simulink model "gm_Copy_of_uz_pmsm_model_9ph_21b_all_double"  (R2022a)
settings: Solver=FixedStepAuto  StartTime=0.0  StopTime=0.8  RelTol=1e-3
PreLoadFcn:
  | uz_pmsm_model_9ph_init_parameter
undefined symbols (not defined in the file or in its folder): a, b, c, friction_coefficient, inertia, k_i_d, k_i_q, k_p_d, k_p_q, Kpd, L_d, L_o1, L_o2, L_q, L_x1, L_x2, L_y1, L_y2, L_zero, polepair, psi_pm, R_1, static_friction_torque, Tnd, ts
libraries: hdlsllib x90, hdlmdlgenlib x21, slpidlib x2, simulink x2, spsAlphaBetaZerotodq0Lib x1, pid_lib x1, spsdq0toAlphaBetaZeroLib x1
(part 2 of 3)

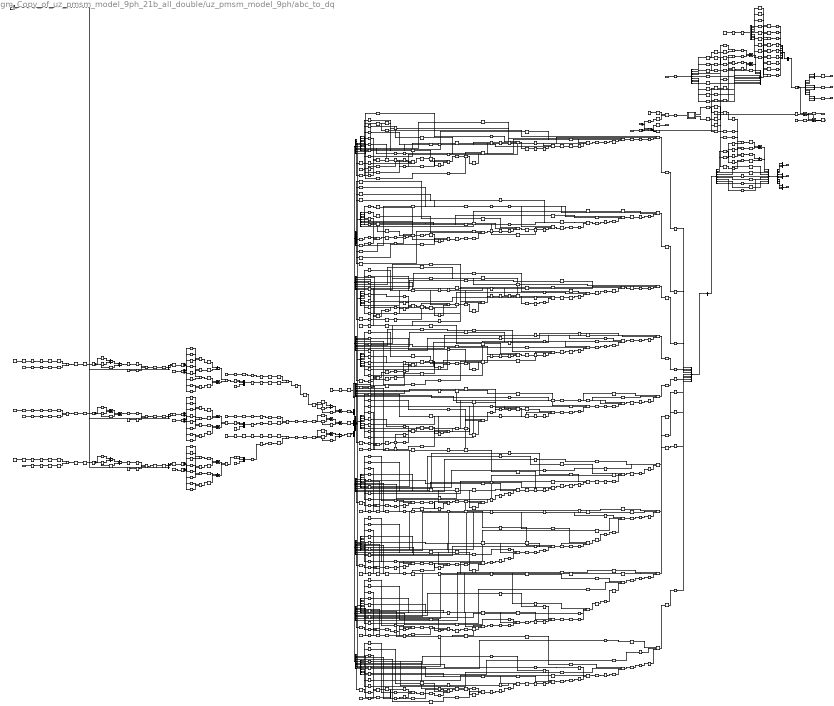
== system gm_Copy_of_uz_pmsm_model_9ph_21b_all_double/uz_pmsm_model_9ph/abc_to_dq ==
  current_in_dq : Inport  OutDataTypeStr=fixdt(1, 25, 12)  PortDimensions=[9]  SampleTime=1e-08
  theta_el1 : Inport  Port=2  OutDataTypeStr=fixdt(1, 18, 14)  PortDimensions=1  SampleTime=1e-08
  trigger_new_values : Inport  Port=3  OutDataTypeStr=boolean  PortDimensions=1  SampleTime=1e-08
  u_abc1_pl : Inport  Port=4  OutDataTypeStr=fixdt(1, 25, 12)  PortDimensions=[3]  SampleTime=1e-08
  u_abc2_pl : Inport  Port=5  OutDataTypeStr=fixdt(1, 25, 12)  PortDimensions=[3]  SampleTime=1e-08
  u_abc3_pl : Inport  Port=6  OutDataTypeStr=fixdt(1, 25, 12)  PortDimensions=[3]  SampleTime=1e-08
  Add : Sum  AccumDataTypeStr=fixdt(1, 26, 12)  OutDataTypeStr=fixdt(1, 25, 12)  SampleTime=1e-08
  Add1 : Sum  Inputs=+-  AccumDataTypeStr=fixdt(1, 26, 12)  OutDataTypeStr=fixdt(1, 25, 12)  SampleTime=1e-08
  Add11 : Sum  AccumDataTypeStr=fixdt(1, 26, 12)  OutDataTypeStr=fixdt(1, 25, 12)  SampleTime=1e-08
  Add2 : Sum  Inputs=+-  AccumDataTypeStr=fixdt(1, 26, 12)  OutDataTypeStr=fixdt(1, 25, 12)  SampleTime=1e-08
  Complex to Real-Imag : ComplexToRealImag  SampleTime=1e-08
  Complex to Real-Imag1 : ComplexToRealImag  SampleTime=1e-08
  Complex to Real-Imag2 : ComplexToRealImag  SampleTime=1e-08
  Constant : Constant  Value=0  OutDataTypeStr=fixdt(1, 25, 12)  SampleTime=1e-08
  Constant1 : Constant  Value="fi(0,1,18,16,\"hex\",\"08000 + 3b619 i\")"  OutDataTypeStr=fixdt(1, 18, 16)  SampleTime=1e-08
  Constant11 : Constant  Value="fi(0,1,18,16,\"hex\",\"08000 + 3b619 i\")"  OutDataTypeStr=fixdt(1, 18, 16)  SampleTime=1e-08
  Constant12 : Constant  Value="fi(0,1,18,16,\"hex\",\"08000 + 3b619 i\")"  OutDataTypeStr=fixdt(1, 18, 16)  SampleTime=1e-08
  Constant13 : Constant  Value=[0.22222137451171875;0;0.22222137451171875;0;0.22222137451171875;0;0.22222137451171875;0;0.111114501953125;-0.111114501953125;0.19245147705078125;0.22222137451171875;0;-0.111114501953125;-0.19245147705078125;-0.111114501953125;0.19245147705078125;0.111114501953125;-0.111114501953125;-0.19245147705078125;0.22222137451171875;0;-0.111114501953125;0.19245147705078125;-0.111114501953125;-0.19245147705078125;0.111114501953125;0.20882415771484375;0.0760040283203125;0.111114501953125;0.19245147705078125;-0.0385894775390625;0.21884918212890625;-0.17023468017578125;0.14284515380859375;-0.111114501953125;-0.17023468017578125;0.14284515380859375;0.111114501953125;0.19245147705078125;0.20882415771484375;-0.0760040283203125;-0.0385894775390625;-0.21884918212890625;-0.111114501953125;-0.0385894775390625;-0.21884918212890625;0.111114501953125;0.19245147705078125;-0.17023468017578125;-0.14284515380859375;0.20882415771484375;0.0760040283203125;-0.111114501953125;0.17023468017578125;0.14284515380859375;-0.111114501953125;0.19245147705078125;-0.20882415771484375;-0.0760040283203125;0.0385894775390625;-0.21884918212890625;0.111114501953125;-0.20882415771484375;0.0760040283203125;-0.111114501953125;0.19245147705078125;0.0385894775390625;0.21884918212890625;0.17023468017578125;0.14284515380859375;0.111114501953125;0.0385894775390625;-0.21884918212890625;-0.111114501953125;0.19245147705078125;0.17023468017578125;-0.14284515380859375;-0.20882415771484375;0.0760040283203125;0.111114501953125]  OutDataTypeStr=fixdt(1, 18, 17)  SampleTime=1e-08
  Constant14 : Constant  Value=[1;-0.5;-0.5;0.939697265625;-0.7660369873046875;-0.17364501953125;0.7660369873046875;-0.939697265625;0.17364501953125;0;0.86602783203125;-0.86602783203125;0.3420257568359375;0.642791748046875;-0.98480224609375;0.642791748046875;0.3420257568359375;-0.98480224609375;1;1;1;0.5;0.5;0.5;-0.5;-0.5;-0.5;0;0;0;0.86602783203125;0.86602783203125;0.86602783203125;0.86602783203125;0.86602783203125;0.86602783203125;1;-0.5;-0.5;-0.17364501953125;0.939697265625;-0.7660369873046875;-0.939697265625;0.17364501953125;0.7660369873046875;0;-0.86602783203125;0.86602783203125;0.98480224609375;-0.3420257568359375;-0.642791748046875;-0.3420257568359375;0.98480224609375;-0.642791748046875;1;-0.5;-0.5;-0.7660369873046875;-0.17364501953125;0.939697265625;0.17364501953125;0.7660369873046875;-0.939697265625;0;0.86602783203125;-0.86602783203125;0.642791748046875;-0.98480224609375;0.3420257568359375;-0.98480224609375;0.642791748046875;0.3420257568359375;1;1;1;-1;-1;-1;1;1;1]  OutDataTypeStr=fixdt(1, 18, 16)  SampleTime=1e-08
  Constant2 : Constant  Value=0  OutDataTypeStr=fixdt(1, 25, 12)  SampleTime=1e-08
  Constant3 : Constant  Value=0  OutDataTypeStr=fixdt(1, 25, 12)  SampleTime=1e-08
  Data Type Conversion28 : DataTypeConversion  OutDataTypeStr=fixdt(1, 25, 12)  RndMeth=Nearest  SampleTime=1e-08  SaturateOnIntegerOverflow=off
  Data Type Conversion28_out1_0_wire : hdlmdlgenlib/Buffer
      settings: SourceProductBaseCode=SL
  Data Type Conversion28_out1_1_wire : hdlmdlgenlib/Buffer
      settings: SourceProductBaseCode=SL
  Delay1 : Delay  DelayLength=double(1)  InitialCondition=0  SampleTime=1e-08
  Delay2 : Delay  DelayLength=double(1)  InitialCondition=0  SampleTime=1e-08
  Delay9 : Delay  DelayLength=double(1)  InitialCondition=0  SampleTime=1e-08
  Delay9_enbsw : Switch  Criteria=u2 ~= 0  Threshold=double(0)  OutDataTypeStr=fixdt(1, 25, 12)  SampleTime=1e-08  SaturateOnIntegerOverflow=off  InputSameDT=off
  Demux1_mux_1 : Mux  Inputs=3
  Demux1_mux_2 : Mux  Inputs=3
  Demux1_mux_3 : Mux  Inputs=3
  Demux_mux_1 : Mux  Inputs=3
  Demux_mux_2 : Mux  Inputs=3
  Demux_mux_3 : Mux  Inputs=3
  Divide{,1..4,11,21,31} (8 alike) : Product  Inputs=**  OutDataTypeStr=fixdt(1, 25, 12)  SampleTime=1e-08
  From{1..2,11,17..18,21,171,181} (8 alike) : hdlmdlgenlib/Buffer
      settings: SourceProductBaseCode=SL
  Gain : Product  Inputs=**  OutDataTypeStr=fixdt(1, 18, 16)  SampleTime=1e-08
  Gain2 : Product  Inputs=**  OutDataTypeStr=fixdt(1, 43, 28)  SampleTime=1e-08
  Gain21 : Product  Inputs=**  OutDataTypeStr=fixdt(1, 43, 28)  SampleTime=1e-08
  Gain22 : Product  Inputs=**  OutDataTypeStr=fixdt(1, 43, 28)  SampleTime=1e-08
  Gain2_const : Constant  Value=0.6666717529296875  OutDataTypeStr=fixdt(1, 18, 16)  SampleTime=1e-08
  Gain2_const1 : Constant  Value=0.6666717529296875  OutDataTypeStr=fixdt(1, 18, 16)  SampleTime=1e-08
  Gain2_const2 : Constant  Value=0.6666717529296875  OutDataTypeStr=fixdt(1, 18, 16)  SampleTime=1e-08
  Gain2_out_dtc : DataTypeConversion  OutDataTypeStr=fixdt(1, 25, 12)  SampleTime=1e-08  RndMeth=Floor
  Gain2_out_dtc1 : DataTypeConversion  OutDataTypeStr=fixdt(1, 25, 12)  SampleTime=1e-08  RndMeth=Floor
  Gain2_out_dtc2 : DataTypeConversion  OutDataTypeStr=fixdt(1, 25, 12)  SampleTime=1e-08  RndMeth=Floor
  Gain4_const : Constant  Value=[1;0;0.5;-0.5;0.86602783203125;0.5;-0.5;-0.86602783203125;0.5]  OutDataTypeStr=fixdt(1, 18, 16)  SampleTime=1e-08
  Gain4_const1 : Constant  Value=[1;-0.5;-0.5;0;0.86602783203125;-0.86602783203125;1;1;1]  OutDataTypeStr=fixdt(1, 18, 16)  SampleTime=1e-08
  Gain4_const2 : Constant  Value=[1;0;0.5;-0.5;0.86602783203125;0.5;-0.5;-0.86602783203125;0.5]  OutDataTypeStr=fixdt(1, 18, 16)  SampleTime=1e-08
  Gain4_const3 : Constant  Value=[1;-0.5;-0.5;0;0.86602783203125;-0.86602783203125;1;1;1]  OutDataTypeStr=fixdt(1, 18, 16)  SampleTime=1e-08
  Gain4_const4 : Constant  Value=[1;0;0.5;-0.5;0.86602783203125;0.5;-0.5;-0.86602783203125;0.5]  OutDataTypeStr=fixdt(1, 18, 16)  SampleTime=1e-08
  Gain4_const5 : Constant  Value=[1;-0.5;-0.5;0;0.86602783203125;-0.86602783203125;1;1;1]  OutDataTypeStr=fixdt(1, 18, 16)  SampleTime=1e-08
  Gain_const : Constant  Value=0.1591548919677734375  OutDataTypeStr=fixdt(1, 18, 19)  SampleTime=1e-08
  Goto15 : hdlmdlgenlib/Buffer
      settings: SourceProductBaseCode=SL
  Goto16 : hdlmdlgenlib/Buffer
      settings: SourceProductBaseCode=SL
  HwModeRegister{,1..302} (303 alike) : Delay  DelayLength=double(1)  InitialCondition=0  SampleTime=1e-08
  MMul_add_01 : Sum  OutDataTypeStr=fixdt(1, 25, 12)  SaturateOnIntegerOverflow=on  SampleTime=1e-08
  MMul_add_011 : Sum  OutDataTypeStr=fixdt(1, 25, 12)  SaturateOnIntegerOverflow=on  SampleTime=1e-08
  MMul_add_012 : Sum  OutDataTypeStr=fixdt(1, 25, 12)  SaturateOnIntegerOverflow=on  SampleTime=1e-08
  MMul_add_013 : Sum  OutDataTypeStr=fixdt(1, 25, 12)  SaturateOnIntegerOverflow=on  SampleTime=1e-08
  MMul_add_014 : Sum  OutDataTypeStr=fixdt(1, 25, 12)  SaturateOnIntegerOverflow=on  SampleTime=1e-08
  MMul_add_015 : Sum  OutDataTypeStr=fixdt(1, 25, 12)  SaturateOnIntegerOverflow=on  SampleTime=1e-08
  MMul_add_{12,121..125} (6 alike) : Sum  OutDataTypeStr=fixdt(1, 25, 12)  SaturateOnIntegerOverflow=on  SampleTime=1e-08
  MMul_dot_product{,1..5} (6 alike) : Product  Inputs=**  OutDataTypeStr=fixdt(1, 43, 28)  SampleTime=1e-08
  MMul_dot_product_out_dtc{,1..5} (6 alike) : DataTypeConversion  OutDataTypeStr=fixdt(1, 25, 12)  SampleTime=1e-08  RndMeth=Floor
  MatrixMultiply_out1_0_wire : hdlmdlgenlib/Buffer
      settings: SourceProductBaseCode=SL
  MatrixMultiply_out1_1_wire : hdlmdlgenlib/Buffer
      settings: SourceProductBaseCode=SL
  PipelineRegister{,1..22,104..119} (39 alike) : Delay  DelayLength=double(1)  InitialCondition=0  SampleTime=1e-08
  PipelineRegister{23..103} (81 alike) : Delay  DelayLength=double(2)  InitialCondition=0  SampleTime=1e-08
  Product{,1..11} (12 alike) : Product  Inputs=**  OutDataTypeStr=fixdt(1, 25, 12)  SampleTime=1e-08
  Product_AC_minus_BD : Sum  Inputs=+-  OutDataTypeStr=fixdt(1, 25, 12)  SampleTime=1e-08
  Product_AC_minus_BD1 : Sum  Inputs=+-  OutDataTypeStr=fixdt(1, 25, 12)  SampleTime=1e-08
  Product_AC_minus_BD2 : Sum  Inputs=+-  OutDataTypeStr=fixdt(1, 25, 12)  SampleTime=1e-08
  Product_AD_plus_BC : Sum  OutDataTypeStr=fixdt(1, 25, 12)  SampleTime=1e-08
  Product_AD_plus_BC1 : Sum  OutDataTypeStr=fixdt(1, 25, 12)  SampleTime=1e-08
  Product_AD_plus_BC2 : Sum  OutDataTypeStr=fixdt(1, 25, 12)  SampleTime=1e-08
  Product_C2ReIm_{1..2,11..12,21..22} (6 alike) : ComplexToRealImag  SampleTime=1e-08
  Product_ReIm2Complex : RealImagToComplex  SampleTime=1e-08
  Product_ReIm2Complex1 : RealImagToComplex  SampleTime=1e-08
  Product_ReIm2Complex2 : RealImagToComplex  SampleTime=1e-08
  Real-Imag to Complex : RealImagToComplex  ConstantPart="fi(0,1,25,12,\"hex\",\"0000000\")"  SampleTime=1e-08
  Real-Imag to Complex1 : RealImagToComplex  ConstantPart="fi(0,1,25,12,\"hex\",\"0000000\")"  SampleTime=1e-08
  Real-Imag to Complex2 : RealImagToComplex  ConstantPart="fi(0,1,25,12,\"hex\",\"0000000\")"  SampleTime=1e-08
  Reshape{,1..5} (6 alike) : Reshape  OutputDimensionality=Column vector (2-D)
  Row2Col_in{0..1,11..15} (7 alike) : Reshape  OutputDimensionality=Column vector (2-D)
  Row2Col_in01 : Reshape  OutputDimensionality=Column vector (2-D)
  Row2Col_in02 : Reshape  OutputDimensionality=Column vector (2-D)
  Row2Col_in03 : Reshape  OutputDimensionality=Column vector (2-D)
  Row2Col_in04 : Reshape  OutputDimensionality=Column vector (2-D)
  Row2Col_in05 : Reshape  OutputDimensionality=Column vector (2-D)
  Sine HDL Optimized : Subsystem  mask(Sine and Cosine HDL optimized block){OutputFormula=sin(2*pi*u) and cos(2*pi*u), NumDataPoints=double(64), TableDataTypeStr=fixdt(0,16,15), SimulateLUTROMDelay=off}
      mask prompts: OutputFormula "Simulink:masks:OutputFormula_MP"; NumDataPoints "HDLShared:hdlshared:CosineHDL_Npts"; TableDataTypeStr "Simulink:blkprm_prompts:TABLE_UNIFIEDDATATYPE"; SimulateLUTROMDelay "HDLShared:hdlshared:CosineHDL_SimulateLUTDelay"
      mask help: Sine and Cosine HDL optimized block using quarter wave symmetry, and HDL friendly settings.
      mask Help: helpview([docroot '/hdlcoder/helptargets.map'],'SineAndCosineHDL_Optimized');
      mask TypeOptions OutputFormula: sin(2*pi*u) | cos(2*pi*u) | exp(j*2*pi*u) | sin(2*pi*u) and cos(2*pi*u)
      mask Display:
      | port_label('input',1,'u')
      | port_label('output',1,'sin(2*pi*u)')
      | port_label('output',2,'cos(2*pi*u)')
      | xpos = 0.35;
      | yoffset = 0.5;
      | if ( SimulateLUTROMDelay )
      |   text(xpos,yoffset,'HDL (Z^{-1})','texmode','on')
      | else
      |    text(xpos,yoffset,'HDL')
      | end
  Switch : Switch  Criteria=u2 ~= 0  Threshold=double(0)  OutDataTypeStr=fixdt(1, 25, 12)  SampleTime=1e-08  SaturateOnIntegerOverflow=off  InputSameDT=off
  Switch1 : Switch  Criteria=u2 ~= 0  Threshold=double(0)  OutDataTypeStr=fixdt(1, 18, 14)  SampleTime=1e-08  SaturateOnIntegerOverflow=off  InputSameDT=off
  Transformation1_out1 : hdlmdlgenlib/Buffer
      settings: SourceProductBaseCode=SL
  Unit Delay : UnitDelay  SampleTime=1e-08
  _adder_MultiplyAdd{,1..80} (81 alike) : hdlsllib/HDL Operations/Multiply-Add  Function=c+(a.*b)  datatype=fixdt(1, 44, 29)  DoSatur=off  FMA=off
      settings: SourceProductBaseCode=SL
  _adder_MultiplyAdd_out_dtc{,1..80} (81 alike) : DataTypeConversion  OutDataTypeStr=fixdt(1, 25, 12)  SampleTime=1e-08  SaturateOnIntegerOverflow=off  RndMeth=Floor
  _bias{,1..8} (9 alike) : Constant  Value=double(0)  OutDataTypeStr=fixdt(1, 25, 12)  SampleTime=1e-08
  abc   to   alpha_beta_0_out1_2_term2 : Terminator
  abc   to   alpha_beta_0_out1_2_term21 : Terminator
  abc   to   alpha_beta_0_out1_2_term22 : Terminator
  delayMatch{,1..2,7,24,41,58,75,92,109,126,143} (12 alike) : Delay  DelayLength=double(6)  InitialCondition=0  SampleTime=1e-08
  delayMatch{10,27,44,61,78,95,112,129,146} (9 alike) : Delay  DelayLength=double(20)  InitialCondition=0  SampleTime=1e-08
  delayMatch{15,32,49,66,83,100,117,134,151} (9 alike) : Delay  DelayLength=double(18)  InitialCondition=0  SampleTime=1e-08
  delayMatch{16,33,50,67,84,101,118,135,152} (9 alike) : Delay  DelayLength=double(29)  InitialCondition=0  SampleTime=1e-08
  delayMatch{17,34,51,68,85,102,119,136,153} (9 alike) : Delay  DelayLength=double(21)  InitialCondition=0  SampleTime=1e-08
  delayMatch{18,35,52,69,86,103,120,137,154,189..192} (13 alike) : Delay  DelayLength=double(32)  InitialCondition=0  SampleTime=1e-08
  delayMatch{19,36,53,70,87,104,121,138,155} (9 alike) : Delay  DelayLength=double(24)  InitialCondition=0  SampleTime=1e-08
  delayMatch{3,20,37,54,71,88,105,122,139} (9 alike) : Delay  DelayLength=double(8)  InitialCondition=0  SampleTime=1e-08
  delayMatch{4,21,38,55,72,89,106,123,140} (9 alike) : Delay  DelayLength=double(11)  InitialCondition=0  SampleTime=1e-08
  delayMatch{5,22,39,56,73,90,107,124,141} (9 alike) : Delay  DelayLength=double(3)  InitialCondition=0  SampleTime=1e-08
  delayMatch{6,23,40,57,74,91,108,125,142} (9 alike) : Delay  DelayLength=double(14)  InitialCondition=0  SampleTime=1e-08
  delayMatch{11,28,45,62,79,96,113,130,147} (9 alike) : Delay  DelayLength=double(12)  InitialCondition=0  SampleTime=1e-08
  delayMatch{8,25,42,59,76,93,110,127,144} (9 alike) : Delay  DelayLength=double(17)  InitialCondition=0  SampleTime=1e-08
  delayMatch{9,26,43,60,77,94,111,128,145} (9 alike) : Delay  DelayLength=double(9)  InitialCondition=0  SampleTime=1e-08
  delayMatch{12,29,46,63,80,97,114,131,148} (9 alike) : Delay  DelayLength=double(23)  InitialCondition=0  SampleTime=1e-08
  delayMatch{13,30,47,64,81,98,115,132,149} (9 alike) : Delay  DelayLength=double(15)  InitialCondition=0  SampleTime=1e-08
  delayMatch{14,31,48,65,82,99,116,133,150} (9 alike) : Delay  DelayLength=double(26)  InitialCondition=0  SampleTime=1e-08
  delayMatch{156..159} (4 alike) : Delay  DelayLength=double(33)  InitialCondition=0  SampleTime=1e-08
  delayMatch{160..170} (11 alike) : Delay  DelayLength=double(2)  InitialCondition=0  SampleTime=1e-08
  delayMatch{171..186} (16 alike) : Delay  DelayLength=double(4)  InitialCondition=0  SampleTime=1e-08
  delayMatch187 : Delay  DelayLength=double(5)  InitialCondition=0  SampleTime=1e-08
  delayMatch188 : Delay  DelayLength=double(5)  InitialCondition=0  SampleTime=1e-08
  delayMatch193 : Delay  DelayLength=double(37)  InitialCondition=0  SampleTime=1e-08
  mux : Mux  Inputs=3
  mux1 : Mux  Inputs=3
  mux2 : Mux  Inputs=3
  mux3 : Mux  Inputs=9
  mux4 : Mux  Inputs=9
  mux5 : Mux  Inputs=9
  reshape_dotProduct{,1..5} (6 alike) : Reshape  OutputDimensionality=Customize  OutputDimensions=[3,3]
  reshape_mmulResult{,1..5} (6 alike) : Reshape  OutputDimensionality=Customize  OutputDimensions=[3,1]
  select_0 : Selector  NumberOfDimensions=2  SampleTime=1e-08  IndexOptions=Index vector (dialog),Select all  Indices=double(1),[]  OutputSizes=1
  select_01 : Selector  NumberOfDimensions=2  SampleTime=1e-08  IndexOptions=Index vector (dialog),Select all  Indices=double(1),[]  OutputSizes=1
  select_02 : Selector  NumberOfDimensions=2  SampleTime=1e-08  IndexOptions=Index vector (dialog),Select all  Indices=double(1),[]  OutputSizes=1
  select_03 : Selector  NumberOfDimensions=2  SampleTime=1e-08  IndexOptions=Index vector (dialog),Select all  Indices=double(1),[]  OutputSizes=1
  select_04 : Selector  NumberOfDimensions=2  SampleTime=1e-08  IndexOptions=Index vector (dialog),Select all  Indices=double(1),[]  OutputSizes=1
  select_05 : Selector  NumberOfDimensions=2  SampleTime=1e-08  IndexOptions=Index vector (dialog),Select all  Indices=double(1),[]  OutputSizes=1
  select_{1,11..15} (6 alike) : Selector  NumberOfDimensions=2  SampleTime=1e-08  IndexOptions=Index vector (dialog),Select all  Indices=double(2),[]  OutputSizes=1
  select_{2,21..25} (6 alike) : Selector  NumberOfDimensions=2  SampleTime=1e-08  IndexOptions=Index vector (dialog),Select all  Indices=double(3),[]  OutputSizes=1
  select_indices0 : Selector  SampleTime=1e-08  IndexOptions=Index vector (dialog)  Indices=double([1 4 7 2 5 8 3 6 9])  OutputSizes=1
  select_indices01 : Selector  SampleTime=1e-08  IndexOptions=Index vector (dialog)  Indices=double([1 4 7 2 5 8 3 6 9])  OutputSizes=1
  select_indices02 : Selector  SampleTime=1e-08  IndexOptions=Index vector (dialog)  Indices=double([1 4 7 2 5 8 3 6 9])  OutputSizes=1
  select_indices03 : Selector  SampleTime=1e-08  IndexOptions=Index vector (dialog)  Indices=double([1 4 7 2 5 8 3 6 9])  OutputSizes=1
  select_indices04 : Selector  SampleTime=1e-08  IndexOptions=Index vector (dialog)  Indices=double([1 4 7 2 5 8 3 6 9])  OutputSizes=1
  select_indices05 : Selector  SampleTime=1e-08  IndexOptions=Index vector (dialog)  Indices=double([1 4 7 2 5 8 3 6 9])  OutputSizes=1
  select_indices{1,11..15} (6 alike) : Selector  SampleTime=1e-08  IndexOptions=Index vector (dialog)  Indices=double([1 2 3 1 2 3 1 2 3])  OutputSizes=1
  stateControl : Constant  OutDataTypeStr=boolean  SampleTime=1e-08
  t{,1,8..9,35..52} (22 alike) : Demux  Outputs=9
  t{10..15} (6 alike) : Reshape  OutputDimensionality=Customize  OutputDimensions=[3,3]
  t16 : Reshape  OutputDimensionality=Customize  OutputDimensions=[9,9]
  t17 : Reshape  OutputDimensionality=Customize  OutputDimensions=[9,9]
  t18 : Math  Operator=transpose
  t19 : Subsystem
  t{2..7} (6 alike) : Demux  Outputs=3
  t20 : Mux  Inputs=9
  t21 : Concatenate  NumInputs=1  Mode=Multidimensional array  ConcatenateDimension=2
  t22 : Math  Operator=transpose
  t23 : Subsystem
  t{24..32} (9 alike) : hdlsllib/HDL Operations/Multiply-Accumulate  opMode=Vector  initValueSetting=Dialog  initValue=0  initValueSetting2=Dialog  initValue2=0  initValueSetting3=Dialog  initValue3=0  num_samples=2  RndMeth2=Floor  RndMeth3=Floor  OutDataTypeStr=fixdt(1, 25, 12)  datatype2=Inherit: Inherit via back propagation  datatype3=Inherit: Inherit via back propagation  validOut=on  endInandOut=on  startOut=on  countOut=on  dim=-1  DoSatur=off  parallel=off
      settings: SourceProductBaseCode=SL
  t33 : Mux  Inputs=9
  t34 : Concatenate  NumInputs=1  Mode=Multidimensional array  ConcatenateDimension=2
  vectorized_in0 : Reshape  OutputDimensionality=Row vector (2-D)
  vectorized_in01 : Reshape  OutputDimensionality=Row vector (2-D)
  vectorized_in02 : Reshape  OutputDimensionality=Row vector (2-D)
  vectorized_in03 : Reshape  OutputDimensionality=Row vector (2-D)
  vectorized_in04 : Reshape  OutputDimensionality=Row vector (2-D)
  vectorized_in05 : Reshape  OutputDimensionality=Row vector (2-D)
  voltage_out_dq_1 : Outport  SampleTime=1e-08
  voltage_out_dq_2 : Outport  Port=2  SampleTime=1e-08
  voltage_out_dq_3 : Outport  Port=3  SampleTime=1e-08
  i_abc_out_axi : Outport  Port=4  SampleTime=1e-08
  I_abc_1 : Outport  Port=5  SampleTime=1e-08
  I_abc_2 : Outport  Port=6  SampleTime=1e-08
  I_abc_3 : Outport  Port=7  SampleTime=1e-08
  theta_el_axi : Outport  Port=8  SampleTime=1e-08
  wires:
  current_in_dq/1 -> Data Type Conversion28/1
  theta_el1/1 -> Delay1/1, Switch1/1
  trigger_new_values/1 -> Unit Delay/1
  u_abc1_pl/1 -> Reshape/1
  u_abc2_pl/1 -> Reshape2/1
  u_abc3_pl/1 -> Reshape4/1
  Delay1/1 -> HwModeRegister278/1
  Demux_mux_1/1 -> voltage_out_dq_1/1
  Demux_mux_2/1 -> voltage_out_dq_2/1
  Demux_mux_3/1 -> voltage_out_dq_3/1
  delayMatch190/1 -> I_abc_1/1
  delayMatch191/1 -> I_abc_2/1
  delayMatch192/1 -> I_abc_3/1
  PipelineRegister107/1 -> Sine HDL Optimized/1(u)
  mux3/1 -> t52/1, t50/1, t48/1, t46/1, t44/1, t42/1, t40/1, t38/1, t36/1
  Sine HDL Optimized/1(x) -> Goto15/1
  Sine HDL Optimized/2(y) -> Goto16/1
  delayMatch189/1 -> i_abc_out_axi/1
  delayMatch193/1 -> theta_el_axi/1
  Transformation1_out1/1 -> t1/1, Switch/1
  delayMatch188/1 -> Switch/2
  Goto15/1 -> From18/1, From1/1, From181/1, From11/1
  Goto16/1 -> From2/1, From17/1, From21/1, From171/1
  Complex to Real-Imag/1 -> mux/1
  Complex to Real-Imag/2 -> mux/2
  Constant/1 -> mux/3
  Constant1/1 -> Product_C2ReIm_2/1
  mux/1 -> Reshape1/1
  Product_ReIm2Complex/1 -> Complex to Real-Imag/1
  Real-Imag to Complex/1 -> Product_C2ReIm_1/1
  Gain2_out_dtc/1 -> t2/1
  reshape_mmulResult/1 -> HwModeRegister271/1
  Reshape/1 -> select_indices1/1
  reshape_mmulResult1/1 -> t5/1
  Reshape1/1 -> select_indices11/1
  Complex to Real-Imag1/1 -> mux1/1
  Complex to Real-Imag1/2 -> mux1/2
  Constant2/1 -> mux1/3
  Constant11/1 -> Product_C2ReIm_21/1
  mux1/1 -> Reshape3/1
  Product_ReIm2Complex1/1 -> Complex to Real-Imag1/1
  Real-Imag to Complex1/1 -> Product_C2ReIm_11/1
  Gain2_out_dtc1/1 -> t3/1
  reshape_mmulResult2/1 -> HwModeRegister273/1
  Reshape2/1 -> select_indices12/1
  reshape_mmulResult3/1 -> t6/1
  Reshape3/1 -> select_indices13/1
  Complex to Real-Imag2/1 -> mux2/1
  Complex to Real-Imag2/2 -> mux2/2
  Constant3/1 -> mux2/3
  Constant12/1 -> Product_C2ReIm_22/1
  mux2/1 -> Reshape5/1
  Product_ReIm2Complex2/1 -> Complex to Real-Imag2/1
  Real-Imag to Complex2/1 -> Product_C2ReIm_12/1
  Gain2_out_dtc2/1 -> t4/1
  reshape_mmulResult4/1 -> HwModeRegister275/1
  Reshape4/1 -> select_indices14/1
  reshape_mmulResult5/1 -> t7/1
  Reshape5/1 -> select_indices15/1
  Add/1 -> mux4/1
  Add1/1 -> mux4/2
  t16/1 -> t18/1
  MatrixMultiply_out1_0_wire/1 -> HwModeRegister1/1, HwModeRegister5/1
  MatrixMultiply_out1_1_wire/1 -> HwModeRegister3/1, HwModeRegister7/1
  delayMatch160/1 -> mux4/3
  delayMatch161/1 -> mux4/4
  delayMatch162/1 -> mux4/5
  delayMatch163/1 -> mux4/6
  delayMatch164/1 -> mux4/7
  delayMatch165/1 -> mux4/8
  delayMatch166/1 -> mux4/9
  PipelineRegister/1 -> Add/1
  PipelineRegister1/1 -> Add/2
  PipelineRegister2/1 -> Add1/2
  PipelineRegister3/1 -> Add1/1
  delayMatch159/1 -> HwModeRegister4/1
  delayMatch156/1 -> HwModeRegister/1
  delayMatch158/1 -> HwModeRegister2/1
  delayMatch157/1 -> HwModeRegister6/1
  t21/1 -> t8/1
  mux4/1 -> t/1
  Add2/1 -> mux5/1
  Add11/1 -> mux5/2
  t17/1 -> t22/1
  Data Type Conversion28/1 -> t9/1
  delayMatch167/1 -> HwModeRegister9/1
  delayMatch169/1 -> HwModeRegister11/1
  delayMatch171/1 -> mux5/3
  delayMatch172/1 -> mux5/4
  delayMatch173/1 -> mux5/5
  delayMatch174/1 -> mux5/6
  delayMatch175/1 -> mux5/7
  delayMatch176/1 -> mux5/8
  delayMatch177/1 -> mux5/9
  PipelineRegister4/1 -> Add2/1
  PipelineRegister5/1 -> Add2/2
  PipelineRegister6/1 -> Add11/1
  PipelineRegister7/1 -> Add11/2
  From11/1 -> HwModeRegister12/1
  From171/1 -> HwModeRegister8/1
  From181/1 -> HwModeRegister10/1
  From21/1 -> HwModeRegister14/1
  t34/1 -> Transformation1_out1/1
  mux5/1 -> t32/2, t31/2, t30/2, t29/2, t28/2, t27/2, t26/2, t25/2, t24/2
  t/1 -> Demux_mux_1/1
  t/2 -> Demux_mux_1/2
  t/3 -> Demux_mux_1/3
  t/4 -> Demux_mux_2/1
  t/5 -> Demux_mux_2/2
  t/6 -> Demux_mux_2/3
  t/7 -> Demux_mux_3/1
  t/8 -> Demux_mux_3/2
  t/9 -> Demux_mux_3/3
  t1/1 -> Demux1_mux_1/1
  t1/2 -> Demux1_mux_1/2
  t1/3 -> Demux1_mux_1/3
  t1/4 -> Demux1_mux_2/1
  t1/5 -> Demux1_mux_2/2
  t1/6 -> Demux1_mux_2/3
  t1/7 -> Demux1_mux_3/1
  t1/8 -> Demux1_mux_3/2
  t1/9 -> Demux1_mux_3/3
  t2/1 -> Real-Imag to Complex/1
  t2/2 -> Real-Imag to Complex/2
  t2/3 -> abc   to   alpha_beta_0_out1_2_term2/1
  t3/1 -> Real-Imag to Complex1/1
  t3/2 -> Real-Imag to Complex1/2
  t3/3 -> abc   to   alpha_beta_0_out1_2_term21/1
  t4/1 -> Real-Imag to Complex2/1
  t4/2 -> Real-Imag to Complex2/2
  t4/3 -> abc   to   alpha_beta_0_out1_2_term22/1
  t5/1 -> mux3/1
  t5/2 -> mux3/2
  t5/3 -> mux3/3
  t6/1 -> mux3/4
  t6/2 -> mux3/5
  t6/3 -> mux3/6
  t7/1 -> mux3/7
  t7/2 -> mux3/8
  t7/3 -> mux3/9
  t8/1 -> MatrixMultiply_out1_0_wire/1
  t8/2 -> MatrixMultiply_out1_1_wire/1
  t8/3 -> delayMatch160/1
  t8/4 -> delayMatch161/1
  t8/5 -> delayMatch162/1
  t8/6 -> delayMatch163/1
  t8/7 -> delayMatch164/1
  t8/8 -> delayMatch165/1
  t8/9 -> delayMatch166/1
  t9/1 -> Data Type Conversion28_out1_0_wire/1
  t9/2 -> Data Type Conversion28_out1_1_wire/1
  t9/3 -> delayMatch171/1
  t9/4 -> delayMatch172/1
  t9/5 -> delayMatch173/1
  t9/6 -> delayMatch174/1
  t9/7 -> delayMatch175/1
  t9/8 -> delayMatch176/1
  t9/9 -> delayMatch177/1
  t10/1 -> vectorized_in0/1
  vectorized_in0/1 -> select_indices0/1
  select_indices0/1 -> Row2Col_in0/1
  select_indices1/1 -> Row2Col_in1/1
  Row2Col_in0/1 -> HwModeRegister16/1
  Row2Col_in1/1 -> HwModeRegister17/1
  MMul_dot_product_out_dtc/1 -> reshape_dotProduct/1
  reshape_dotProduct/1 -> select_2/1, select_1/1, select_0/1
  select_0/1 -> MMul_add_01/1
  select_1/1 -> MMul_add_01/2
  MMul_add_01/1 -> MMul_add_12/1
  select_2/1 -> MMul_add_12/2
  MMul_add_12/1 -> reshape_mmulResult/1
  Gain4_const/1 -> t10/1
  t11/1 -> vectorized_in01/1
  vectorized_in01/1 -> select_indices01/1
  select_indices01/1 -> Row2Col_in01/1
  select_indices11/1 -> Row2Col_in11/1
  delayMatch/1 -> HwModeRegister18/1
  Row2Col_in11/1 -> HwModeRegister19/1
  MMul_dot_product_out_dtc1/1 -> reshape_dotProduct1/1
  reshape_dotProduct1/1 -> select_21/1, select_11/1, select_01/1
  select_01/1 -> MMul_add_011/1
  select_11/1 -> MMul_add_011/2
  MMul_add_011/1 -> MMul_add_121/1
  select_21/1 -> MMul_add_121/2
  MMul_add_121/1 -> reshape_mmulResult1/1
  Gain4_const1/1 -> t11/1
  t12/1 -> vectorized_in02/1
  vectorized_in02/1 -> select_indices02/1
  select_indices02/1 -> Row2Col_in02/1
  select_indices12/1 -> Row2Col_in12/1
  Row2Col_in02/1 -> HwModeRegister20/1
  Row2Col_in12/1 -> HwModeRegister21/1
  MMul_dot_product_out_dtc2/1 -> reshape_dotProduct2/1
  reshape_dotProduct2/1 -> select_22/1, select_12/1, select_02/1
  select_02/1 -> MMul_add_012/1
  select_12/1 -> MMul_add_012/2
  MMul_add_012/1 -> MMul_add_122/1
  select_22/1 -> MMul_add_122/2
  MMul_add_122/1 -> reshape_mmulResult2/1
  Gain4_const2/1 -> t12/1
  t13/1 -> vectorized_in03/1
  vectorized_in03/1 -> select_indices03/1
  select_indices03/1 -> Row2Col_in03/1
  select_indices13/1 -> Row2Col_in13/1
  delayMatch1/1 -> HwModeRegister22/1
  Row2Col_in13/1 -> HwModeRegister23/1
  MMul_dot_product_out_dtc3/1 -> reshape_dotProduct3/1
  reshape_dotProduct3/1 -> select_23/1, select_13/1, select_03/1
  select_03/1 -> MMul_add_013/1
  select_13/1 -> MMul_add_013/2
  MMul_add_013/1 -> MMul_add_123/1
  select_23/1 -> MMul_add_123/2
  MMul_add_123/1 -> reshape_mmulResult3/1
  Gain4_const3/1 -> t13/1
  t14/1 -> vectorized_in04/1
  vectorized_in04/1 -> select_indices04/1
  select_indices04/1 -> Row2Col_in04/1
  select_indices14/1 -> Row2Col_in14/1
  Row2Col_in04/1 -> HwModeRegister24/1
  Row2Col_in14/1 -> HwModeRegister25/1
  MMul_dot_product_out_dtc4/1 -> reshape_dotProduct4/1
  reshape_dotProduct4/1 -> select_24/1, select_14/1, select_04/1
  select_04/1 -> MMul_add_014/1
  select_14/1 -> MMul_add_014/2
  MMul_add_014/1 -> MMul_add_124/1
  select_24/1 -> MMul_add_124/2
  MMul_add_124/1 -> reshape_mmulResult4/1
  Gain4_const4/1 -> t14/1
  t15/1 -> vectorized_in05/1
  vectorized_in05/1 -> select_indices05/1
  select_indices05/1 -> Row2Col_in05/1
  select_indices15/1 -> Row2Col_in15/1
  delayMatch2/1 -> HwModeRegister26/1
  Row2Col_in15/1 -> HwModeRegister27/1
  MMul_dot_product_out_dtc5/1 -> reshape_dotProduct5/1
  reshape_dotProduct5/1 -> select_25/1, select_15/1, select_05/1
  select_05/1 -> MMul_add_015/1
  select_15/1 -> MMul_add_015/2
  MMul_add_015/1 -> MMul_add_125/1
  select_25/1 -> MMul_add_125/2
  MMul_add_125/1 -> reshape_mmulResult5/1
  Gain4_const5/1 -> t15/1
  Constant13/1 -> t16/1
  Constant14/1 -> t17/1
  t18/1 -> t19/1(in0)
  t19/1(out0) -> t35/1
  t19/2(out1) -> t37/1
  t19/3(out2) -> t39/1
  t19/4(out3) -> t41/1
  t19/5(out4) -> t43/1
  t19/6(out5) -> t45/1
  t19/7(out6) -> t47/1
  t19/8(out7) -> t49/1
  t19/9(out8) -> t51/1
  _adder_MultiplyAdd_out_dtc8/1 -> t20/1
  _adder_MultiplyAdd_out_dtc17/1 -> t20/2
  _adder_MultiplyAdd_out_dtc26/1 -> t20/3
  _adder_MultiplyAdd_out_dtc35/1 -> t20/4
  _adder_MultiplyAdd_out_dtc44/1 -> t20/5
  _adder_MultiplyAdd_out_dtc53/1 -> t20/6
  _adder_MultiplyAdd_out_dtc62/1 -> t20/7
  _adder_MultiplyAdd_out_dtc71/1 -> t20/8
  _adder_MultiplyAdd_out_dtc80/1 -> t20/9
  t20/1 -> t21/1
  t22/1 -> t23/1(in0)
  delayMatch178/1 -> t24/1
  delayMatch179/1 -> t25/1
  delayMatch180/1 -> t26/1
  delayMatch181/1 -> t27/1
  delayMatch182/1 -> t28/1
  delayMatch183/1 -> t29/1
  delayMatch184/1 -> t30/1
  delayMatch185/1 -> t31/1
  delayMatch186/1 -> t32/1
  t33/1 -> t34/1
  _bias/1 -> HwModeRegister30/1
  delayMatch3/1 -> HwModeRegister28/1
  t36/1 -> HwModeRegister29/1
  delayMatch4/1 -> HwModeRegister31/1
  delayMatch5/1 -> HwModeRegister32/1
  _adder_MultiplyAdd_out_dtc/1 -> HwModeRegister33/1
  delayMatch6/1 -> HwModeRegister34/1
  delayMatch7/1 -> HwModeRegister35/1
  _adder_MultiplyAdd_out_dtc1/1 -> HwModeRegister36/1
  delayMatch8/1 -> HwModeRegister37/1
  delayMatch9/1 -> HwModeRegister38/1
  _adder_MultiplyAdd_out_dtc2/1 -> HwModeRegister39/1
  delayMatch10/1 -> HwModeRegister40/1
  delayMatch11/1 -> HwModeRegister41/1
  _adder_MultiplyAdd_out_dtc3/1 -> HwModeRegister42/1
  delayMatch12/1 -> HwModeRegister43/1
  delayMatch13/1 -> HwModeRegister44/1
  _adder_MultiplyAdd_out_dtc4/1 -> HwModeRegister45/1
  delayMatch14/1 -> HwModeRegister46/1
  delayMatch15/1 -> HwModeRegister47/1
  _adder_MultiplyAdd_out_dtc5/1 -> HwModeRegister48/1
  delayMatch16/1 -> HwModeRegister49/1
  delayMatch17/1 -> HwModeRegister50/1
  _adder_MultiplyAdd_out_dtc6/1 -> HwModeRegister51/1
  delayMatch18/1 -> HwModeRegister52/1
  delayMatch19/1 -> HwModeRegister53/1
  _adder_MultiplyAdd_out_dtc7/1 -> HwModeRegister54/1
  _bias1/1 -> HwModeRegister57/1
  delayMatch20/1 -> HwModeRegister55/1
  t38/1 -> HwModeRegister56/1
  delayMatch21/1 -> HwModeRegister58/1
  delayMatch22/1 -> HwModeRegister59/1
  _adder_MultiplyAdd_out_dtc9/1 -> HwModeRegister60/1
  delayMatch23/1 -> HwModeRegister61/1
  delayMatch24/1 -> HwModeRegister62/1
  _adder_MultiplyAdd_out_dtc10/1 -> HwModeRegister63/1
  delayMatch25/1 -> HwModeRegister64/1
  delayMatch26/1 -> HwModeRegister65/1
  _adder_MultiplyAdd_out_dtc11/1 -> HwModeRegister66/1
  delayMatch27/1 -> HwModeRegister67/1
  delayMatch28/1 -> HwModeRegister68/1
  _adder_MultiplyAdd_out_dtc12/1 -> HwModeRegister69/1
  delayMatch29/1 -> HwModeRegister70/1
  delayMatch30/1 -> HwModeRegister71/1
  _adder_MultiplyAdd_out_dtc13/1 -> HwModeRegister72/1
  delayMatch31/1 -> HwModeRegister73/1
  delayMatch32/1 -> HwModeRegister74/1
  _adder_MultiplyAdd_out_dtc14/1 -> HwModeRegister75/1
  delayMatch33/1 -> HwModeRegister76/1
  delayMatch34/1 -> HwModeRegister77/1
  _adder_MultiplyAdd_out_dtc15/1 -> HwModeRegister78/1
  delayMatch35/1 -> HwModeRegister79/1
  delayMatch36/1 -> HwModeRegister80/1
  _adder_MultiplyAdd_out_dtc16/1 -> HwModeRegister81/1
  _bias2/1 -> HwModeRegister84/1
  delayMatch37/1 -> HwModeRegister82/1
  t40/1 -> HwModeRegister83/1
  delayMatch38/1 -> HwModeRegister85/1
  delayMatch39/1 -> HwModeRegister86/1
  _adder_MultiplyAdd_out_dtc18/1 -> HwModeRegister87/1
  delayMatch40/1 -> HwModeRegister88/1
  delayMatch41/1 -> HwModeRegister89/1
  _adder_MultiplyAdd_out_dtc19/1 -> HwModeRegister90/1
  delayMatch42/1 -> HwModeRegister91/1
  delayMatch43/1 -> HwModeRegister92/1
  _adder_MultiplyAdd_out_dtc20/1 -> HwModeRegister93/1
  delayMatch44/1 -> HwModeRegister94/1
  delayMatch45/1 -> HwModeRegister95/1
  _adder_MultiplyAdd_out_dtc21/1 -> HwModeRegister96/1
  delayMatch46/1 -> HwModeRegister97/1
  delayMatch47/1 -> HwModeRegister98/1
  _adder_MultiplyAdd_out_dtc22/1 -> HwModeRegister99/1
  delayMatch48/1 -> HwModeRegister100/1
  delayMatch49/1 -> HwModeRegister101/1
  _adder_MultiplyAdd_out_dtc23/1 -> HwModeRegister102/1
  delayMatch50/1 -> HwModeRegister103/1
  delayMatch51/1 -> HwModeRegister104/1
  _adder_MultiplyAdd_out_dtc24/1 -> HwModeRegister105/1
  delayMatch52/1 -> HwModeRegister106/1
  delayMatch53/1 -> HwModeRegister107/1
  _adder_MultiplyAdd_out_dtc25/1 -> HwModeRegister108/1
  _bias3/1 -> HwModeRegister111/1
  delayMatch54/1 -> HwModeRegister109/1
  t42/1 -> HwModeRegister110/1
  delayMatch55/1 -> HwModeRegister112/1
  delayMatch56/1 -> HwModeRegister113/1
  _adder_MultiplyAdd_out_dtc27/1 -> HwModeRegister114/1
  delayMatch57/1 -> HwModeRegister115/1
  delayMatch58/1 -> HwModeRegister116/1
  _adder_MultiplyAdd_out_dtc28/1 -> HwModeRegister117/1
  delayMatch59/1 -> HwModeRegister118/1
  delayMatch60/1 -> HwModeRegister119/1
  _adder_MultiplyAdd_out_dtc29/1 -> HwModeRegister120/1
  delayMatch61/1 -> HwModeRegister121/1
  delayMatch62/1 -> HwModeRegister122/1
  _adder_MultiplyAdd_out_dtc30/1 -> HwModeRegister123/1
  delayMatch63/1 -> HwModeRegister124/1
  delayMatch64/1 -> HwModeRegister125/1
  _adder_MultiplyAdd_out_dtc31/1 -> HwModeRegister126/1
  delayMatch65/1 -> HwModeRegister127/1
  delayMatch66/1 -> HwModeRegister128/1
  _adder_MultiplyAdd_out_dtc32/1 -> HwModeRegister129/1
  delayMatch67/1 -> HwModeRegister130/1
  delayMatch68/1 -> HwModeRegister131/1
  _adder_MultiplyAdd_out_dtc33/1 -> HwModeRegister132/1
  delayMatch69/1 -> HwModeRegister133/1
  delayMatch70/1 -> HwModeRegister134/1
  _adder_MultiplyAdd_out_dtc34/1 -> HwModeRegister135/1
  _bias4/1 -> HwModeRegister138/1
  delayMatch71/1 -> HwModeRegister136/1
  t44/1 -> HwModeRegister137/1
  delayMatch72/1 -> HwModeRegister139/1
  delayMatch73/1 -> HwModeRegister140/1
  _adder_MultiplyAdd_out_dtc36/1 -> HwModeRegister141/1
  delayMatch74/1 -> HwModeRegister142/1
  delayMatch75/1 -> HwModeRegister143/1
  _adder_MultiplyAdd_out_dtc37/1 -> HwModeRegister144/1
  delayMatch76/1 -> HwModeRegister145/1
  delayMatch77/1 -> HwModeRegister146/1
  _adder_MultiplyAdd_out_dtc38/1 -> HwModeRegister147/1
  delayMatch78/1 -> HwModeRegister148/1
  delayMatch79/1 -> HwModeRegister149/1
  _adder_MultiplyAdd_out_dtc39/1 -> HwModeRegister150/1
  delayMatch80/1 -> HwModeRegister151/1
  delayMatch81/1 -> HwModeRegister152/1
  _adder_MultiplyAdd_out_dtc40/1 -> HwModeRegister153/1
  delayMatch82/1 -> HwModeRegister154/1
  delayMatch83/1 -> HwModeRegister155/1
  _adder_MultiplyAdd_out_dtc41/1 -> HwModeRegister156/1
  delayMatch84/1 -> HwModeRegister157/1
  delayMatch85/1 -> HwModeRegister158/1
  _adder_MultiplyAdd_out_dtc42/1 -> HwModeRegister159/1
  delayMatch86/1 -> HwModeRegister160/1
  delayMatch87/1 -> HwModeRegister161/1
  _adder_MultiplyAdd_out_dtc43/1 -> HwModeRegister162/1
  _bias5/1 -> HwModeRegister165/1
  delayMatch88/1 -> HwModeRegister163/1
  t46/1 -> HwModeRegister164/1
  delayMatch89/1 -> HwModeRegister166/1
  delayMatch90/1 -> HwModeRegister167/1
  _adder_MultiplyAdd_out_dtc45/1 -> HwModeRegister168/1
  delayMatch91/1 -> HwModeRegister169/1
  delayMatch92/1 -> HwModeRegister170/1
  _adder_MultiplyAdd_out_dtc46/1 -> HwModeRegister171/1
  delayMatch93/1 -> HwModeRegister172/1
  delayMatch94/1 -> HwModeRegister173/1
  _adder_MultiplyAdd_out_dtc47/1 -> HwModeRegister174/1
  delayMatch95/1 -> HwModeRegister175/1
  delayMatch96/1 -> HwModeRegister176/1
  _adder_MultiplyAdd_out_dtc48/1 -> HwModeRegister177/1
  delayMatch97/1 -> HwModeRegister178/1
  delayMatch98/1 -> HwModeRegister179/1
  _adder_MultiplyAdd_out_dtc49/1 -> HwModeRegister180/1
  delayMatch99/1 -> HwModeRegister181/1
  delayMatch100/1 -> HwModeRegister182/1
  _adder_MultiplyAdd_out_dtc50/1 -> HwModeRegister183/1
  delayMatch101/1 -> HwModeRegister184/1
  delayMatch102/1 -> HwModeRegister185/1
  _adder_MultiplyAdd_out_dtc51/1 -> HwModeRegister186/1
  delayMatch103/1 -> HwModeRegister187/1
  delayMatch104/1 -> HwModeRegister188/1
  _adder_MultiplyAdd_out_dtc52/1 -> HwModeRegister189/1
  _bias6/1 -> HwModeRegister192/1
  delayMatch105/1 -> HwModeRegister190/1
  t48/1 -> HwModeRegister191/1
  delayMatch106/1 -> HwModeRegister193/1
  delayMatch107/1 -> HwModeRegister194/1
  _adder_MultiplyAdd_out_dtc54/1 -> HwModeRegister195/1
  delayMatch108/1 -> HwModeRegister196/1
  delayMatch109/1 -> HwModeRegister197/1
  _adder_MultiplyAdd_out_dtc55/1 -> HwModeRegister198/1
  delayMatch110/1 -> HwModeRegister199/1
  delayMatch111/1 -> HwModeRegister200/1
  _adder_MultiplyAdd_out_dtc56/1 -> HwModeRegister201/1
  delayMatch112/1 -> HwModeRegister202/1
  delayMatch113/1 -> HwModeRegister203/1
  _adder_MultiplyAdd_out_dtc57/1 -> HwModeRegister204/1
  delayMatch114/1 -> HwModeRegister205/1
  delayMatch115/1 -> HwModeRegister206/1
  _adder_MultiplyAdd_out_dtc58/1 -> HwModeRegister207/1
  delayMatch116/1 -> HwModeRegister208/1
  delayMatch117/1 -> HwModeRegister209/1
  _adder_MultiplyAdd_out_dtc59/1 -> HwModeRegister210/1
  delayMatch118/1 -> HwModeRegister211/1
  delayMatch119/1 -> HwModeRegister212/1
  _adder_MultiplyAdd_out_dtc60/1 -> HwModeRegister213/1
  delayMatch120/1 -> HwModeRegister214/1
  delayMatch121/1 -> HwModeRegister215/1
  _adder_MultiplyAdd_out_dtc61/1 -> HwModeRegister216/1
  _bias7/1 -> HwModeRegister219/1
  delayMatch122/1 -> HwModeRegister217/1
  t50/1 -> HwModeRegister218/1
  delayMatch123/1 -> HwModeRegister220/1
  delayMatch124/1 -> HwModeRegister221/1
  _adder_MultiplyAdd_out_dtc63/1 -> HwModeRegister222/1
  delayMatch125/1 -> HwModeRegister223/1
  delayMatch126/1 -> HwModeRegister224/1
  _adder_MultiplyAdd_out_dtc64/1 -> HwModeRegister225/1
  delayMatch127/1 -> HwModeRegister226/1
  delayMatch128/1 -> HwModeRegister227/1
  _adder_MultiplyAdd_out_dtc65/1 -> HwModeRegister228/1
  delayMatch129/1 -> HwModeRegister229/1
  delayMatch130/1 -> HwModeRegister230/1
  _adder_MultiplyAdd_out_dtc66/1 -> HwModeRegister231/1
  delayMatch131/1 -> HwModeRegister232/1
  delayMatch132/1 -> HwModeRegister233/1
  _adder_MultiplyAdd_out_dtc67/1 -> HwModeRegister234/1
  delayMatch133/1 -> HwModeRegister235/1
  delayMatch134/1 -> HwModeRegister236/1
  _adder_MultiplyAdd_out_dtc68/1 -> HwModeRegister237/1
  delayMatch135/1 -> HwModeRegister238/1
  delayMatch136/1 -> HwModeRegister239/1
  _adder_MultiplyAdd_out_dtc69/1 -> HwModeRegister240/1
  delayMatch137/1 -> HwModeRegister241/1
  delayMatch138/1 -> HwModeRegister242/1
  _adder_MultiplyAdd_out_dtc70/1 -> HwModeRegister243/1
  _bias8/1 -> HwModeRegister246/1
  delayMatch139/1 -> HwModeRegister244/1
  t52/1 -> HwModeRegister245/1
  delayMatch140/1 -> HwModeRegister247/1
  delayMatch141/1 -> HwModeRegister248/1
  _adder_MultiplyAdd_out_dtc72/1 -> HwModeRegister249/1
  delayMatch142/1 -> HwModeRegister250/1
  delayMatch143/1 -> HwModeRegister251/1
  _adder_MultiplyAdd_out_dtc73/1 -> HwModeRegister252/1
  delayMatch144/1 -> HwModeRegister253/1
  delayMatch145/1 -> HwModeRegister254/1
  _adder_MultiplyAdd_out_dtc74/1 -> HwModeRegister255/1
  delayMatch146/1 -> HwModeRegister256/1
  delayMatch147/1 -> HwModeRegister257/1
  _adder_MultiplyAdd_out_dtc75/1 -> HwModeRegister258/1
  delayMatch148/1 -> HwModeRegister259/1
  delayMatch149/1 -> HwModeRegister260/1
  _adder_MultiplyAdd_out_dtc76/1 -> HwModeRegister261/1
  delayMatch150/1 -> HwModeRegister262/1
  delayMatch151/1 -> HwModeRegister263/1
  _adder_MultiplyAdd_out_dtc77/1 -> HwModeRegister264/1
  delayMatch152/1 -> HwModeRegister265/1
  delayMatch153/1 -> HwModeRegister266/1
  _adder_MultiplyAdd_out_dtc78/1 -> HwModeRegister267/1
  delayMatch154/1 -> HwModeRegister268/1
  delayMatch155/1 -> HwModeRegister269/1
  _adder_MultiplyAdd_out_dtc79/1 -> HwModeRegister270/1
  Gain2_const/1 -> HwModeRegister272/1
  Gain2_const1/1 -> HwModeRegister274/1
  Gain2_const2/1 -> HwModeRegister276/1
  Gain_const/1 -> HwModeRegister277/1
  delayMatch187/1 -> Delay9_enbsw/2
  Row2Col_in01/1 -> delayMatch/1
  Row2Col_in03/1 -> delayMatch1/1
  Row2Col_in05/1 -> delayMatch2/1
  t35/1 -> delayMatch3/1
  t35/2 -> delayMatch4/1
  t36/2 -> delayMatch5/1
  t35/3 -> delayMatch6/1
  t36/3 -> delayMatch7/1
  t35/4 -> delayMatch8/1
  t36/4 -> delayMatch9/1
  t35/5 -> delayMatch10/1
  t36/5 -> delayMatch11/1
  t35/6 -> delayMatch12/1
  t36/6 -> delayMatch13/1
  t35/7 -> delayMatch14/1
  t36/7 -> delayMatch15/1
  t35/8 -> delayMatch16/1
  t36/8 -> delayMatch17/1
  t35/9 -> delayMatch18/1
  t36/9 -> delayMatch19/1
  t37/1 -> delayMatch20/1
  t37/2 -> delayMatch21/1
  t38/2 -> delayMatch22/1
  t37/3 -> delayMatch23/1
  t38/3 -> delayMatch24/1
  t37/4 -> delayMatch25/1
  t38/4 -> delayMatch26/1
  t37/5 -> delayMatch27/1
  t38/5 -> delayMatch28/1
  t37/6 -> delayMatch29/1
  t38/6 -> delayMatch30/1
  t37/7 -> delayMatch31/1
  t38/7 -> delayMatch32/1
  t37/8 -> delayMatch33/1
  t38/8 -> delayMatch34/1
  t37/9 -> delayMatch35/1
  t38/9 -> delayMatch36/1
  t39/1 -> delayMatch37/1
  t39/2 -> delayMatch38/1
  t40/2 -> delayMatch39/1
  t39/3 -> delayMatch40/1
  t40/3 -> delayMatch41/1
  t39/4 -> delayMatch42/1
  t40/4 -> delayMatch43/1
  t39/5 -> delayMatch44/1
  t40/5 -> delayMatch45/1
  t39/6 -> delayMatch46/1
  t40/6 -> delayMatch47/1
  t39/7 -> delayMatch48/1
  t40/7 -> delayMatch49/1
  t39/8 -> delayMatch50/1
  t40/8 -> delayMatch51/1
  t39/9 -> delayMatch52/1
  t40/9 -> delayMatch53/1
  t41/1 -> delayMatch54/1
  t41/2 -> delayMatch55/1
  t42/2 -> delayMatch56/1
  t41/3 -> delayMatch57/1
  t42/3 -> delayMatch58/1
  t41/4 -> delayMatch59/1
  t42/4 -> delayMatch60/1
  t41/5 -> delayMatch61/1
  t42/5 -> delayMatch62/1
  t41/6 -> delayMatch63/1
  t42/6 -> delayMatch64/1
  t41/7 -> delayMatch65/1
  t42/7 -> delayMatch66/1
  t41/8 -> delayMatch67/1
  t42/8 -> delayMatch68/1
  t41/9 -> delayMatch69/1
  t42/9 -> delayMatch70/1
  t43/1 -> delayMatch71/1
  t43/2 -> delayMatch72/1
  t44/2 -> delayMatch73/1
  t43/3 -> delayMatch74/1
  t44/3 -> delayMatch75/1
  t43/4 -> delayMatch76/1
  t44/4 -> delayMatch77/1
  t43/5 -> delayMatch78/1
  t44/5 -> delayMatch79/1
  t43/6 -> delayMatch80/1
  t44/6 -> delayMatch81/1
  t43/7 -> delayMatch82/1
  t44/7 -> delayMatch83/1
  t43/8 -> delayMatch84/1
  t44/8 -> delayMatch85/1
  t43/9 -> delayMatch86/1
  t44/9 -> delayMatch87/1
  t45/1 -> delayMatch88/1
  t45/2 -> delayMatch89/1
  t46/2 -> delayMatch90/1
  t45/3 -> delayMatch91/1
  t46/3 -> delayMatch92/1
  t45/4 -> delayMatch93/1
  t46/4 -> delayMatch94/1
  t45/5 -> delayMatch95/1
  t46/5 -> delayMatch96/1
  t45/6 -> delayMatch97/1
  t46/6 -> delayMatch98/1
  t45/7 -> delayMatch99/1
  t46/7 -> delayMatch100/1
  t45/8 -> delayMatch101/1
  t46/8 -> delayMatch102/1
  t45/9 -> delayMatch103/1
  t46/9 -> delayMatch104/1
  t47/1 -> delayMatch105/1
  t47/2 -> delayMatch106/1
  t48/2 -> delayMatch107/1
  t47/3 -> delayMatch108/1
  t48/3 -> delayMatch109/1
  t47/4 -> delayMatch110/1
  t48/4 -> delayMatch111/1
  t47/5 -> delayMatch112/1
  t48/5 -> delayMatch113/1
  t47/6 -> delayMatch114/1
  t48/6 -> delayMatch115/1
  t47/7 -> delayMatch116/1
  t48/7 -> delayMatch117/1
  t47/8 -> delayMatch118/1
  t48/8 -> delayMatch119/1
  t47/9 -> delayMatch120/1
  t48/9 -> delayMatch121/1
  t49/1 -> delayMatch122/1
  t49/2 -> delayMatch123/1
  t50/2 -> delayMatch124/1
  t49/3 -> delayMatch125/1
  t50/3 -> delayMatch126/1
  t49/4 -> delayMatch127/1
  t50/4 -> delayMatch128/1
  t49/5 -> delayMatch129/1
  t50/5 -> delayMatch130/1
  t49/6 -> delayMatch131/1
  t50/6 -> delayMatch132/1
  t49/7 -> delayMatch133/1
  t50/7 -> delayMatch134/1
  t49/8 -> delayMatch135/1
  t50/8 -> delayMatch136/1
  t49/9 -> delayMatch137/1
  t50/9 -> delayMatch138/1
  t51/1 -> delayMatch139/1
  t51/2 -> delayMatch140/1
  t52/2 -> delayMatch141/1
  t51/3 -> delayMatch142/1
  t52/3 -> delayMatch143/1
  t51/4 -> delayMatch144/1
  t52/4 -> delayMatch145/1
  t51/5 -> delayMatch146/1
  t52/5 -> delayMatch147/1
  t51/6 -> delayMatch148/1
  t52/6 -> delayMatch149/1
  t51/7 -> delayMatch150/1
  t52/7 -> delayMatch151/1
  t51/8 -> delayMatch152/1
  t52/8 -> delayMatch153/1
  t51/9 -> delayMatch154/1
  t52/9 -> delayMatch155/1
  From17/1 -> delayMatch156/1
  From2/1 -> delayMatch157/1
  From18/1 -> delayMatch158/1
  From1/1 -> delayMatch159/1
  delayMatch168/1 -> HwModeRegister13/1
  Data Type Conversion28_out1_0_wire/1 -> delayMatch168/1, delayMatch167/1
  delayMatch170/1 -> HwModeRegister15/1
  Data Type Conversion28_out1_1_wire/1 -> delayMatch170/1, delayMatch169/1
  t23/1(out0) -> delayMatch178/1
  t23/2(out1) -> delayMatch179/1
  t23/3(out2) -> delayMatch180/1
  t23/4(out3) -> delayMatch181/1
  t23/5(out4) -> delayMatch182/1
  t23/6(out5) -> delayMatch183/1
  t23/7(out6) -> delayMatch184/1
  t23/8(out7) -> delayMatch185/1
  t23/9(out8) -> delayMatch186/1
  stateControl/1 -> delayMatch187/1
  Unit Delay/1 -> delayMatch188/1, Switch1/2
  Demux1_mux_1/1 -> delayMatch190/1
  Demux1_mux_2/1 -> delayMatch191/1
  Demux1_mux_3/1 -> delayMatch192/1
  Switch1/1 -> delayMatch193/1, Delay2/1
  Switch/1 -> delayMatch189/1, Delay9_enbsw/1
  Product_C2ReIm_1/1 -> HwModeRegister279/1, HwModeRegister281/1
  Product_C2ReIm_1/2 -> HwModeRegister283/1, HwModeRegister285/1
  Product_C2ReIm_2/1 -> HwModeRegister280/1, HwModeRegister286/1
  Product_C2ReIm_2/2 -> HwModeRegister282/1, HwModeRegister284/1
  PipelineRegister108/1 -> Product_AC_minus_BD/1
  PipelineRegister109/1 -> Product_AD_plus_BC/1
  PipelineRegister110/1 -> Product_AC_minus_BD/2
  PipelineRegister111/1 -> Product_AD_plus_BC/2
  Product_AC_minus_BD/1 -> Product_ReIm2Complex/1
  Product_AD_plus_BC/1 -> Product_ReIm2Complex/2
  Product_C2ReIm_11/1 -> HwModeRegister287/1, HwModeRegister289/1
  Product_C2ReIm_11/2 -> HwModeRegister291/1, HwModeRegister293/1
  Product_C2ReIm_21/1 -> HwModeRegister288/1, HwModeRegister294/1
  Product_C2ReIm_21/2 -> HwModeRegister290/1, HwModeRegister292/1
  PipelineRegister112/1 -> Product_AC_minus_BD1/1
  PipelineRegister113/1 -> Product_AD_plus_BC1/1
  PipelineRegister114/1 -> Product_AC_minus_BD1/2
  PipelineRegister115/1 -> Product_AD_plus_BC1/2
  Product_AC_minus_BD1/1 -> Product_ReIm2Complex1/1
  Product_AD_plus_BC1/1 -> Product_ReIm2Complex1/2
  Product_C2ReIm_12/1 -> HwModeRegister295/1, HwModeRegister297/1
  Product_C2ReIm_12/2 -> HwModeRegister299/1, HwModeRegister301/1
  Product_C2ReIm_22/1 -> HwModeRegister296/1, HwModeRegister302/1
  Product_C2ReIm_22/2 -> HwModeRegister298/1, HwModeRegister300/1
  PipelineRegister116/1 -> Product_AC_minus_BD2/1
  PipelineRegister117/1 -> Product_AD_plus_BC2/1
  PipelineRegister118/1 -> Product_AC_minus_BD2/2
  PipelineRegister119/1 -> Product_AD_plus_BC2/2
  Product_AC_minus_BD2/1 -> Product_ReIm2Complex2/1
  Product_AD_plus_BC2/1 -> Product_ReIm2Complex2/2
  PipelineRegister8/1 -> MMul_dot_product_out_dtc/1
  PipelineRegister9/1 -> MMul_dot_product_out_dtc1/1
  PipelineRegister10/1 -> MMul_dot_product_out_dtc2/1
  PipelineRegister11/1 -> MMul_dot_product_out_dtc3/1
  PipelineRegister12/1 -> MMul_dot_product_out_dtc4/1
  PipelineRegister13/1 -> MMul_dot_product_out_dtc5/1
  PipelineRegister23/1 -> _adder_MultiplyAdd_out_dtc/1
  PipelineRegister24/1 -> _adder_MultiplyAdd_out_dtc1/1
  PipelineRegister25/1 -> _adder_MultiplyAdd_out_dtc2/1
  PipelineRegister26/1 -> _adder_MultiplyAdd_out_dtc3/1
  PipelineRegister27/1 -> _adder_MultiplyAdd_out_dtc4/1
  PipelineRegister28/1 -> _adder_MultiplyAdd_out_dtc5/1
  PipelineRegister29/1 -> _adder_MultiplyAdd_out_dtc6/1
  PipelineRegister30/1 -> _adder_MultiplyAdd_out_dtc7/1
  PipelineRegister31/1 -> _adder_MultiplyAdd_out_dtc8/1
  PipelineRegister32/1 -> _adder_MultiplyAdd_out_dtc9/1
  PipelineRegister33/1 -> _adder_MultiplyAdd_out_dtc10/1
  PipelineRegister34/1 -> _adder_MultiplyAdd_out_dtc11/1
  PipelineRegister35/1 -> _adder_MultiplyAdd_out_dtc12/1
  PipelineRegister36/1 -> _adder_MultiplyAdd_out_dtc13/1
  PipelineRegister37/1 -> _adder_MultiplyAdd_out_dtc14/1
  PipelineRegister38/1 -> _adder_MultiplyAdd_out_dtc15/1
  PipelineRegister39/1 -> _adder_MultiplyAdd_out_dtc16/1
  PipelineRegister40/1 -> _adder_MultiplyAdd_out_dtc17/1
  PipelineRegister41/1 -> _adder_MultiplyAdd_out_dtc18/1
  PipelineRegister42/1 -> _adder_MultiplyAdd_out_dtc19/1
  PipelineRegister43/1 -> _adder_MultiplyAdd_out_dtc20/1
  PipelineRegister44/1 -> _adder_MultiplyAdd_out_dtc21/1
  PipelineRegister45/1 -> _adder_MultiplyAdd_out_dtc22/1
  PipelineRegister46/1 -> _adder_MultiplyAdd_out_dtc23/1
  PipelineRegister47/1 -> _adder_MultiplyAdd_out_dtc24/1
  PipelineRegister48/1 -> _adder_MultiplyAdd_out_dtc25/1
  PipelineRegister49/1 -> _adder_MultiplyAdd_out_dtc26/1
  PipelineRegister50/1 -> _adder_MultiplyAdd_out_dtc27/1
  PipelineRegister51/1 -> _adder_MultiplyAdd_out_dtc28/1
  PipelineRegister52/1 -> _adder_MultiplyAdd_out_dtc29/1
  PipelineRegister53/1 -> _adder_MultiplyAdd_out_dtc30/1
  PipelineRegister54/1 -> _adder_MultiplyAdd_out_dtc31/1
  PipelineRegister55/1 -> _adder_MultiplyAdd_out_dtc32/1
  PipelineRegister56/1 -> _adder_MultiplyAdd_out_dtc33/1
  PipelineRegister57/1 -> _adder_MultiplyAdd_out_dtc34/1
  PipelineRegister58/1 -> _adder_MultiplyAdd_out_dtc35/1
  PipelineRegister59/1 -> _adder_MultiplyAdd_out_dtc36/1
  PipelineRegister60/1 -> _adder_MultiplyAdd_out_dtc37/1
  PipelineRegister61/1 -> _adder_MultiplyAdd_out_dtc38/1
  PipelineRegister62/1 -> _adder_MultiplyAdd_out_dtc39/1
  PipelineRegister63/1 -> _adder_MultiplyAdd_out_dtc40/1
  PipelineRegister64/1 -> _adder_MultiplyAdd_out_dtc41/1
  PipelineRegister65/1 -> _adder_MultiplyAdd_out_dtc42/1
  PipelineRegister66/1 -> _adder_MultiplyAdd_out_dtc43/1
  PipelineRegister67/1 -> _adder_MultiplyAdd_out_dtc44/1
  PipelineRegister68/1 -> _adder_MultiplyAdd_out_dtc45/1
  PipelineRegister69/1 -> _adder_MultiplyAdd_out_dtc46/1
  PipelineRegister70/1 -> _adder_MultiplyAdd_out_dtc47/1
  PipelineRegister71/1 -> _adder_MultiplyAdd_out_dtc48/1
  PipelineRegister72/1 -> _adder_MultiplyAdd_out_dtc49/1
  PipelineRegister73/1 -> _adder_MultiplyAdd_out_dtc50/1
  PipelineRegister74/1 -> _adder_MultiplyAdd_out_dtc51/1
  PipelineRegister75/1 -> _adder_MultiplyAdd_out_dtc52/1
  PipelineRegister76/1 -> _adder_MultiplyAdd_out_dtc53/1
  PipelineRegister77/1 -> _adder_MultiplyAdd_out_dtc54/1
  PipelineRegister78/1 -> _adder_MultiplyAdd_out_dtc55/1
  PipelineRegister79/1 -> _adder_MultiplyAdd_out_dtc56/1
  PipelineRegister80/1 -> _adder_MultiplyAdd_out_dtc57/1
  PipelineRegister81/1 -> _adder_MultiplyAdd_out_dtc58/1
  PipelineRegister82/1 -> _adder_MultiplyAdd_out_dtc59/1
  PipelineRegister83/1 -> _adder_MultiplyAdd_out_dtc60/1
  PipelineRegister84/1 -> _adder_MultiplyAdd_out_dtc61/1
  PipelineRegister85/1 -> _adder_MultiplyAdd_out_dtc62/1
  PipelineRegister86/1 -> _adder_MultiplyAdd_out_dtc63/1
  PipelineRegister87/1 -> _adder_MultiplyAdd_out_dtc64/1
  PipelineRegister88/1 -> _adder_MultiplyAdd_out_dtc65/1
  PipelineRegister89/1 -> _adder_MultiplyAdd_out_dtc66/1
  PipelineRegister90/1 -> _adder_MultiplyAdd_out_dtc67/1
  PipelineRegister91/1 -> _adder_MultiplyAdd_out_dtc68/1
  PipelineRegister92/1 -> _adder_MultiplyAdd_out_dtc69/1
  PipelineRegister93/1 -> _adder_MultiplyAdd_out_dtc70/1
  PipelineRegister94/1 -> _adder_MultiplyAdd_out_dtc71/1
  PipelineRegister95/1 -> _adder_MultiplyAdd_out_dtc72/1
  PipelineRegister96/1 -> _adder_MultiplyAdd_out_dtc73/1
  PipelineRegister97/1 -> _adder_MultiplyAdd_out_dtc74/1
  PipelineRegister98/1 -> _adder_MultiplyAdd_out_dtc75/1
  PipelineRegister99/1 -> _adder_MultiplyAdd_out_dtc76/1
  PipelineRegister100/1 -> _adder_MultiplyAdd_out_dtc77/1
  PipelineRegister101/1 -> _adder_MultiplyAdd_out_dtc78/1
  PipelineRegister102/1 -> _adder_MultiplyAdd_out_dtc79/1
  PipelineRegister103/1 -> _adder_MultiplyAdd_out_dtc80/1
  PipelineRegister104/1 -> Gain2_out_dtc/1
  PipelineRegister105/1 -> Gain2_out_dtc1/1
  PipelineRegister106/1 -> Gain2_out_dtc2/1
  PipelineRegister14/1 -> t33/1
  PipelineRegister15/1 -> t33/2
  PipelineRegister16/1 -> t33/3
  PipelineRegister17/1 -> t33/4
  PipelineRegister18/1 -> t33/5
  PipelineRegister19/1 -> t33/6
  PipelineRegister20/1 -> t33/7
  PipelineRegister21/1 -> t33/8
  PipelineRegister22/1 -> t33/9
  Delay9_enbsw/1 -> Delay9/1
  Delay9/1 -> Switch/3, Delay9_enbsw/3
  Delay2/1 -> Switch1/3
  Divide/1 -> PipelineRegister/1
  HwModeRegister/1 -> Divide/1
  HwModeRegister1/1 -> Divide/2
  Divide1/1 -> PipelineRegister1/1
  HwModeRegister2/1 -> Divide1/1
  HwModeRegister3/1 -> Divide1/2
  Divide2/1 -> PipelineRegister2/1
  HwModeRegister4/1 -> Divide2/1
  HwModeRegister5/1 -> Divide2/2
  Divide3/1 -> PipelineRegister3/1
  HwModeRegister6/1 -> Divide3/1
  HwModeRegister7/1 -> Divide3/2
  Divide4/1 -> PipelineRegister4/1
  HwModeRegister8/1 -> Divide4/1
  HwModeRegister9/1 -> Divide4/2
  Divide11/1 -> PipelineRegister5/1
  HwModeRegister10/1 -> Divide11/1
  HwModeRegister11/1 -> Divide11/2
  Divide21/1 -> PipelineRegister6/1
  HwModeRegister12/1 -> Divide21/1
  HwModeRegister13/1 -> Divide21/2
  Divide31/1 -> PipelineRegister7/1
  HwModeRegister14/1 -> Divide31/1
  HwModeRegister15/1 -> Divide31/2
  MMul_dot_product/1 -> PipelineRegister8/1
  HwModeRegister16/1 -> MMul_dot_product/1
  HwModeRegister17/1 -> MMul_dot_product/2
  MMul_dot_product1/1 -> PipelineRegister9/1
  HwModeRegister18/1 -> MMul_dot_product1/1
  HwModeRegister19/1 -> MMul_dot_product1/2
  MMul_dot_product2/1 -> PipelineRegister10/1
  HwModeRegister20/1 -> MMul_dot_product2/1
  HwModeRegister21/1 -> MMul_dot_product2/2
  MMul_dot_product3/1 -> PipelineRegister11/1
  HwModeRegister22/1 -> MMul_dot_product3/1
  HwModeRegister23/1 -> MMul_dot_product3/2
  MMul_dot_product4/1 -> PipelineRegister12/1
  HwModeRegister24/1 -> MMul_dot_product4/1
  HwModeRegister25/1 -> MMul_dot_product4/2
  MMul_dot_product5/1 -> PipelineRegister13/1
  HwModeRegister26/1 -> MMul_dot_product5/1
  HwModeRegister27/1 -> MMul_dot_product5/2
  t24/1 -> PipelineRegister14/1
  t25/1 -> PipelineRegister15/1
  t26/1 -> PipelineRegister16/1
  t27/1 -> PipelineRegister17/1
  t28/1 -> PipelineRegister18/1
  t29/1 -> PipelineRegister19/1
  t30/1 -> PipelineRegister20/1
  t31/1 -> PipelineRegister21/1
  t32/1 -> PipelineRegister22/1
  _adder_MultiplyAdd/1 -> PipelineRegister23/1
  HwModeRegister28/1 -> _adder_MultiplyAdd/1
  HwModeRegister29/1 -> _adder_MultiplyAdd/2
  HwModeRegister30/1 -> _adder_MultiplyAdd/3
  _adder_MultiplyAdd1/1 -> PipelineRegister24/1
  HwModeRegister31/1 -> _adder_MultiplyAdd1/1
  HwModeRegister32/1 -> _adder_MultiplyAdd1/2
  HwModeRegister33/1 -> _adder_MultiplyAdd1/3
  _adder_MultiplyAdd2/1 -> PipelineRegister25/1
  HwModeRegister34/1 -> _adder_MultiplyAdd2/1
  HwModeRegister35/1 -> _adder_MultiplyAdd2/2
  HwModeRegister36/1 -> _adder_MultiplyAdd2/3
  _adder_MultiplyAdd3/1 -> PipelineRegister26/1
  HwModeRegister37/1 -> _adder_MultiplyAdd3/1
  HwModeRegister38/1 -> _adder_MultiplyAdd3/2
  HwModeRegister39/1 -> _adder_MultiplyAdd3/3
  _adder_MultiplyAdd4/1 -> PipelineRegister27/1
  HwModeRegister40/1 -> _adder_MultiplyAdd4/1
  HwModeRegister41/1 -> _adder_MultiplyAdd4/2
  HwModeRegister42/1 -> _adder_MultiplyAdd4/3
  _adder_MultiplyAdd5/1 -> PipelineRegister28/1
  HwModeRegister43/1 -> _adder_MultiplyAdd5/1
  HwModeRegister44/1 -> _adder_MultiplyAdd5/2
  HwModeRegister45/1 -> _adder_MultiplyAdd5/3
  _adder_MultiplyAdd6/1 -> PipelineRegister29/1
  HwModeRegister46/1 -> _adder_MultiplyAdd6/1
  HwModeRegister47/1 -> _adder_MultiplyAdd6/2
  HwModeRegister48/1 -> _adder_MultiplyAdd6/3
  _adder_MultiplyAdd7/1 -> PipelineRegister30/1
  HwModeRegister49/1 -> _adder_MultiplyAdd7/1
  HwModeRegister50/1 -> _adder_MultiplyAdd7/2
  HwModeRegister51/1 -> _adder_MultiplyAdd7/3
  _adder_MultiplyAdd8/1 -> PipelineRegister31/1
  HwModeRegister52/1 -> _adder_MultiplyAdd8/1
  HwModeRegister53/1 -> _adder_MultiplyAdd8/2
  HwModeRegister54/1 -> _adder_MultiplyAdd8/3
  _adder_MultiplyAdd9/1 -> PipelineRegister32/1
  HwModeRegister55/1 -> _adder_MultiplyAdd9/1
  HwModeRegister56/1 -> _adder_MultiplyAdd9/2
  HwModeRegister57/1 -> _adder_MultiplyAdd9/3
  _adder_MultiplyAdd10/1 -> PipelineRegister33/1
  HwModeRegister58/1 -> _adder_MultiplyAdd10/1
  HwModeRegister59/1 -> _adder_MultiplyAdd10/2
  HwModeRegister60/1 -> _adder_MultiplyAdd10/3
  _adder_MultiplyAdd11/1 -> PipelineRegister34/1
  HwModeRegister61/1 -> _adder_MultiplyAdd11/1
  HwModeRegister62/1 -> _adder_MultiplyAdd11/2
  HwModeRegister63/1 -> _adder_MultiplyAdd11/3
  _adder_MultiplyAdd12/1 -> PipelineRegister35/1
  HwModeRegister64/1 -> _adder_MultiplyAdd12/1
  HwModeRegister65/1 -> _adder_MultiplyAdd12/2
  HwModeRegister66/1 -> _adder_MultiplyAdd12/3
  _adder_MultiplyAdd13/1 -> PipelineRegister36/1
  HwModeRegister67/1 -> _adder_MultiplyAdd13/1
  HwModeRegister68/1 -> _adder_MultiplyAdd13/2
  HwModeRegister69/1 -> _adder_MultiplyAdd13/3
  _adder_MultiplyAdd14/1 -> PipelineRegister37/1
  HwModeRegister70/1 -> _adder_MultiplyAdd14/1
  HwModeRegister71/1 -> _adder_MultiplyAdd14/2
  HwModeRegister72/1 -> _adder_MultiplyAdd14/3
  _adder_MultiplyAdd15/1 -> PipelineRegister38/1
  HwModeRegister73/1 -> _adder_MultiplyAdd15/1
  HwModeRegister74/1 -> _adder_MultiplyAdd15/2
  HwModeRegister75/1 -> _adder_MultiplyAdd15/3
  _adder_MultiplyAdd16/1 -> PipelineRegister39/1
  HwModeRegister76/1 -> _adder_MultiplyAdd16/1
  HwModeRegister77/1 -> _adder_MultiplyAdd16/2
  HwModeRegister78/1 -> _adder_MultiplyAdd16/3
  _adder_MultiplyAdd17/1 -> PipelineRegister40/1
  HwModeRegister79/1 -> _adder_MultiplyAdd17/1
  HwModeRegister80/1 -> _adder_MultiplyAdd17/2
  HwModeRegister81/1 -> _adder_MultiplyAdd17/3
  _adder_MultiplyAdd18/1 -> PipelineRegister41/1
  HwModeRegister82/1 -> _adder_MultiplyAdd18/1
  HwModeRegister83/1 -> _adder_MultiplyAdd18/2
  HwModeRegister84/1 -> _adder_MultiplyAdd18/3
  _adder_MultiplyAdd19/1 -> PipelineRegister42/1
  HwModeRegister85/1 -> _adder_MultiplyAdd19/1
  HwModeRegister86/1 -> _adder_MultiplyAdd19/2
  HwModeRegister87/1 -> _adder_MultiplyAdd19/3
  _adder_MultiplyAdd20/1 -> PipelineRegister43/1
  HwModeRegister88/1 -> _adder_MultiplyAdd20/1
  HwModeRegister89/1 -> _adder_MultiplyAdd20/2
  HwModeRegister90/1 -> _adder_MultiplyAdd20/3
  _adder_MultiplyAdd21/1 -> PipelineRegister44/1
  HwModeRegister91/1 -> _adder_MultiplyAdd21/1
  HwModeRegister92/1 -> _adder_MultiplyAdd21/2
  HwModeRegister93/1 -> _adder_MultiplyAdd21/3
  _adder_MultiplyAdd22/1 -> PipelineRegister45/1
  HwModeRegister94/1 -> _adder_MultiplyAdd22/1
  HwModeRegister95/1 -> _adder_MultiplyAdd22/2
  HwModeRegister96/1 -> _adder_MultiplyAdd22/3
  _adder_MultiplyAdd23/1 -> PipelineRegister46/1
  HwModeRegister97/1 -> _adder_MultiplyAdd23/1
  HwModeRegister98/1 -> _adder_MultiplyAdd23/2
  HwModeRegister99/1 -> _adder_MultiplyAdd23/3
  _adder_MultiplyAdd24/1 -> PipelineRegister47/1
  HwModeRegister100/1 -> _adder_MultiplyAdd24/1
  HwModeRegister101/1 -> _adder_MultiplyAdd24/2
  HwModeRegister102/1 -> _adder_MultiplyAdd24/3
  _adder_MultiplyAdd25/1 -> PipelineRegister48/1
  HwModeRegister103/1 -> _adder_MultiplyAdd25/1
  HwModeRegister104/1 -> _adder_MultiplyAdd25/2
  HwModeRegister105/1 -> _adder_MultiplyAdd25/3
  _adder_MultiplyAdd26/1 -> PipelineRegister49/1
  HwModeRegister106/1 -> _adder_MultiplyAdd26/1
  HwModeRegister107/1 -> _adder_MultiplyAdd26/2
  HwModeRegister108/1 -> _adder_MultiplyAdd26/3
  _adder_MultiplyAdd27/1 -> PipelineRegister50/1
  HwModeRegister109/1 -> _adder_MultiplyAdd27/1
  HwModeRegister110/1 -> _adder_MultiplyAdd27/2
  HwModeRegister111/1 -> _adder_MultiplyAdd27/3
  _adder_MultiplyAdd28/1 -> PipelineRegister51/1
  HwModeRegister112/1 -> _adder_MultiplyAdd28/1
  HwModeRegister113/1 -> _adder_MultiplyAdd28/2
  HwModeRegister114/1 -> _adder_MultiplyAdd28/3
  _adder_MultiplyAdd29/1 -> PipelineRegister52/1
  HwModeRegister115/1 -> _adder_MultiplyAdd29/1
  HwModeRegister116/1 -> _adder_MultiplyAdd29/2
  HwModeRegister117/1 -> _adder_MultiplyAdd29/3
  _adder_MultiplyAdd30/1 -> PipelineRegister53/1
  HwModeRegister118/1 -> _adder_MultiplyAdd30/1
  HwModeRegister119/1 -> _adder_MultiplyAdd30/2
  HwModeRegister120/1 -> _adder_MultiplyAdd30/3
  _adder_MultiplyAdd31/1 -> PipelineRegister54/1
  HwModeRegister121/1 -> _adder_MultiplyAdd31/1
  HwModeRegister122/1 -> _adder_MultiplyAdd31/2
  HwModeRegister123/1 -> _adder_MultiplyAdd31/3
  _adder_MultiplyAdd32/1 -> PipelineRegister55/1
  HwModeRegister124/1 -> _adder_MultiplyAdd32/1
  HwModeRegister125/1 -> _adder_MultiplyAdd32/2
  HwModeRegister126/1 -> _adder_MultiplyAdd32/3
  _adder_MultiplyAdd33/1 -> PipelineRegister56/1
  HwModeRegister127/1 -> _adder_MultiplyAdd33/1
  HwModeRegister128/1 -> _adder_MultiplyAdd33/2
  HwModeRegister129/1 -> _adder_MultiplyAdd33/3
  _adder_MultiplyAdd34/1 -> PipelineRegister57/1
  HwModeRegister130/1 -> _adder_MultiplyAdd34/1
  HwModeRegister131/1 -> _adder_MultiplyAdd34/2
  HwModeRegister132/1 -> _adder_MultiplyAdd34/3
  _adder_MultiplyAdd35/1 -> PipelineRegister58/1
  HwModeRegister133/1 -> _adder_MultiplyAdd35/1
  HwModeRegister134/1 -> _adder_MultiplyAdd35/2
  HwModeRegister135/1 -> _adder_MultiplyAdd35/3
  _adder_MultiplyAdd36/1 -> PipelineRegister59/1
  HwModeRegister136/1 -> _adder_MultiplyAdd36/1
  HwModeRegister137/1 -> _adder_MultiplyAdd36/2
  HwModeRegister138/1 -> _adder_MultiplyAdd36/3
  _adder_MultiplyAdd37/1 -> PipelineRegister60/1
  HwModeRegister139/1 -> _adder_MultiplyAdd37/1
  HwModeRegister140/1 -> _adder_MultiplyAdd37/2
  HwModeRegister141/1 -> _adder_MultiplyAdd37/3
  _adder_MultiplyAdd38/1 -> PipelineRegister61/1
  HwModeRegister142/1 -> _adder_MultiplyAdd38/1
  HwModeRegister143/1 -> _adder_MultiplyAdd38/2
  HwModeRegister144/1 -> _adder_MultiplyAdd38/3
  _adder_MultiplyAdd39/1 -> PipelineRegister62/1
  HwModeRegister145/1 -> _adder_MultiplyAdd39/1
  HwModeRegister146/1 -> _adder_MultiplyAdd39/2
  HwModeRegister147/1 -> _adder_MultiplyAdd39/3
  _adder_MultiplyAdd40/1 -> PipelineRegister63/1
  HwModeRegister148/1 -> _adder_MultiplyAdd40/1
  HwModeRegister149/1 -> _adder_MultiplyAdd40/2
  HwModeRegister150/1 -> _adder_MultiplyAdd40/3
  _adder_MultiplyAdd41/1 -> PipelineRegister64/1
  HwModeRegister151/1 -> _adder_MultiplyAdd41/1
  HwModeRegister152/1 -> _adder_MultiplyAdd41/2
  HwModeRegister153/1 -> _adder_MultiplyAdd41/3
  _adder_MultiplyAdd42/1 -> PipelineRegister65/1
  HwModeRegister154/1 -> _adder_MultiplyAdd42/1
  HwModeRegister155/1 -> _adder_MultiplyAdd42/2
  HwModeRegister156/1 -> _adder_MultiplyAdd42/3
  _adder_MultiplyAdd43/1 -> PipelineRegister66/1
  HwModeRegister157/1 -> _adder_MultiplyAdd43/1
  HwModeRegister158/1 -> _adder_MultiplyAdd43/2
  HwModeRegister159/1 -> _adder_MultiplyAdd43/3
  _adder_MultiplyAdd44/1 -> PipelineRegister67/1
  HwModeRegister160/1 -> _adder_MultiplyAdd44/1
  HwModeRegister161/1 -> _adder_MultiplyAdd44/2
  HwModeRegister162/1 -> _adder_MultiplyAdd44/3
  _adder_MultiplyAdd45/1 -> PipelineRegister68/1
  HwModeRegister163/1 -> _adder_MultiplyAdd45/1
  HwModeRegister164/1 -> _adder_MultiplyAdd45/2
  HwModeRegister165/1 -> _adder_MultiplyAdd45/3
  _adder_MultiplyAdd46/1 -> PipelineRegister69/1
  HwModeRegister166/1 -> _adder_MultiplyAdd46/1
  HwModeRegister167/1 -> _adder_MultiplyAdd46/2
  HwModeRegister168/1 -> _adder_MultiplyAdd46/3
  _adder_MultiplyAdd47/1 -> PipelineRegister70/1
  HwModeRegister169/1 -> _adder_MultiplyAdd47/1
  HwModeRegister170/1 -> _adder_MultiplyAdd47/2
  HwModeRegister171/1 -> _adder_MultiplyAdd47/3
  _adder_MultiplyAdd48/1 -> PipelineRegister71/1
  HwModeRegister172/1 -> _adder_MultiplyAdd48/1
  HwModeRegister173/1 -> _adder_MultiplyAdd48/2
  HwModeRegister174/1 -> _adder_MultiplyAdd48/3
  _adder_MultiplyAdd49/1 -> PipelineRegister72/1
  HwModeRegister175/1 -> _adder_MultiplyAdd49/1
  HwModeRegister176/1 -> _adder_MultiplyAdd49/2
  HwModeRegister177/1 -> _adder_MultiplyAdd49/3
  _adder_MultiplyAdd50/1 -> PipelineRegister73/1
  HwModeRegister178/1 -> _adder_MultiplyAdd50/1
  HwModeRegister179/1 -> _adder_MultiplyAdd50/2
  HwModeRegister180/1 -> _adder_MultiplyAdd50/3
  _adder_MultiplyAdd51/1 -> PipelineRegister74/1
  HwModeRegister181/1 -> _adder_MultiplyAdd51/1
  HwModeRegister182/1 -> _adder_MultiplyAdd51/2
  HwModeRegister183/1 -> _adder_MultiplyAdd51/3
  _adder_MultiplyAdd52/1 -> PipelineRegister75/1
  HwModeRegister184/1 -> _adder_MultiplyAdd52/1
  HwModeRegister185/1 -> _adder_MultiplyAdd52/2
  HwModeRegister186/1 -> _adder_MultiplyAdd52/3
  _adder_MultiplyAdd53/1 -> PipelineRegister76/1
  HwModeRegister187/1 -> _adder_MultiplyAdd53/1
  HwModeRegister188/1 -> _adder_MultiplyAdd53/2
  HwModeRegister189/1 -> _adder_MultiplyAdd53/3
  _adder_MultiplyAdd54/1 -> PipelineRegister77/1
  HwModeRegister190/1 -> _adder_MultiplyAdd54/1
  HwModeRegister191/1 -> _adder_MultiplyAdd54/2
  HwModeRegister192/1 -> _adder_MultiplyAdd54/3
  _adder_MultiplyAdd55/1 -> PipelineRegister78/1
  HwModeRegister193/1 -> _adder_MultiplyAdd55/1
  HwModeRegister194/1 -> _adder_MultiplyAdd55/2
  HwModeRegister195/1 -> _adder_MultiplyAdd55/3
  _adder_MultiplyAdd56/1 -> PipelineRegister79/1
  HwModeRegister196/1 -> _adder_MultiplyAdd56/1
  HwModeRegister197/1 -> _adder_MultiplyAdd56/2
  HwModeRegister198/1 -> _adder_MultiplyAdd56/3
  _adder_MultiplyAdd57/1 -> PipelineRegister80/1
  HwModeRegister199/1 -> _adder_MultiplyAdd57/1
  HwModeRegister200/1 -> _adder_MultiplyAdd57/2
  HwModeRegister201/1 -> _adder_MultiplyAdd57/3
  _adder_MultiplyAdd58/1 -> PipelineRegister81/1
  HwModeRegister202/1 -> _adder_MultiplyAdd58/1
  HwModeRegister203/1 -> _adder_MultiplyAdd58/2
  HwModeRegister204/1 -> _adder_MultiplyAdd58/3
  _adder_MultiplyAdd59/1 -> PipelineRegister82/1
  HwModeRegister205/1 -> _adder_MultiplyAdd59/1
  HwModeRegister206/1 -> _adder_MultiplyAdd59/2
  HwModeRegister207/1 -> _adder_MultiplyAdd59/3
  _adder_MultiplyAdd60/1 -> PipelineRegister83/1
  HwModeRegister208/1 -> _adder_MultiplyAdd60/1
  HwModeRegister209/1 -> _adder_MultiplyAdd60/2
  HwModeRegister210/1 -> _adder_MultiplyAdd60/3
  _adder_MultiplyAdd61/1 -> PipelineRegister84/1
  HwModeRegister211/1 -> _adder_MultiplyAdd61/1
  HwModeRegister212/1 -> _adder_MultiplyAdd61/2
  HwModeRegister213/1 -> _adder_MultiplyAdd61/3
  _adder_MultiplyAdd62/1 -> PipelineRegister85/1
  HwModeRegister214/1 -> _adder_MultiplyAdd62/1
  HwModeRegister215/1 -> _adder_MultiplyAdd62/2
  HwModeRegister216/1 -> _adder_MultiplyAdd62/3
  _adder_MultiplyAdd63/1 -> PipelineRegister86/1
  HwModeRegister217/1 -> _adder_MultiplyAdd63/1
  HwModeRegister218/1 -> _adder_MultiplyAdd63/2
  HwModeRegister219/1 -> _adder_MultiplyAdd63/3
  _adder_MultiplyAdd64/1 -> PipelineRegister87/1
  HwModeRegister220/1 -> _adder_MultiplyAdd64/1
  HwModeRegister221/1 -> _adder_MultiplyAdd64/2
  HwModeRegister222/1 -> _adder_MultiplyAdd64/3
  _adder_MultiplyAdd65/1 -> PipelineRegister88/1
  HwModeRegister223/1 -> _adder_MultiplyAdd65/1
  HwModeRegister224/1 -> _adder_MultiplyAdd65/2
  HwModeRegister225/1 -> _adder_MultiplyAdd65/3
  _adder_MultiplyAdd66/1 -> PipelineRegister89/1
  HwModeRegister226/1 -> _adder_MultiplyAdd66/1
  HwModeRegister227/1 -> _adder_MultiplyAdd66/2
  HwModeRegister228/1 -> _adder_MultiplyAdd66/3
  _adder_MultiplyAdd67/1 -> PipelineRegister90/1
  HwModeRegister229/1 -> _adder_MultiplyAdd67/1
  HwModeRegister230/1 -> _adder_MultiplyAdd67/2
  HwModeRegister231/1 -> _adder_MultiplyAdd67/3
  _adder_MultiplyAdd68/1 -> PipelineRegister91/1
  HwModeRegister232/1 -> _adder_MultiplyAdd68/1
  HwModeRegister233/1 -> _adder_MultiplyAdd68/2
  HwModeRegister234/1 -> _adder_MultiplyAdd68/3
  _adder_MultiplyAdd69/1 -> PipelineRegister92/1
  HwModeRegister235/1 -> _adder_MultiplyAdd69/1
  HwModeRegister236/1 -> _adder_MultiplyAdd69/2
  HwModeRegister237/1 -> _adder_MultiplyAdd69/3
  _adder_MultiplyAdd70/1 -> PipelineRegister93/1
  HwModeRegister238/1 -> _adder_MultiplyAdd70/1
  HwModeRegister239/1 -> _adder_MultiplyAdd70/2
  HwModeRegister240/1 -> _adder_MultiplyAdd70/3
  _adder_MultiplyAdd71/1 -> PipelineRegister94/1
  HwModeRegister241/1 -> _adder_MultiplyAdd71/1
  HwModeRegister242/1 -> _adder_MultiplyAdd71/2
  HwModeRegister243/1 -> _adder_MultiplyAdd71/3
  _adder_MultiplyAdd72/1 -> PipelineRegister95/1
  HwModeRegister244/1 -> _adder_MultiplyAdd72/1
  HwModeRegister245/1 -> _adder_MultiplyAdd72/2
  HwModeRegister246/1 -> _adder_MultiplyAdd72/3
  _adder_MultiplyAdd73/1 -> PipelineRegister96/1
  HwModeRegister247/1 -> _adder_MultiplyAdd73/1
  HwModeRegister248/1 -> _adder_MultiplyAdd73/2
  HwModeRegister249/1 -> _adder_MultiplyAdd73/3
  _adder_MultiplyAdd74/1 -> PipelineRegister97/1
  HwModeRegister250/1 -> _adder_MultiplyAdd74/1
  HwModeRegister251/1 -> _adder_MultiplyAdd74/2
  HwModeRegister252/1 -> _adder_MultiplyAdd74/3
  _adder_MultiplyAdd75/1 -> PipelineRegister98/1
  HwModeRegister253/1 -> _adder_MultiplyAdd75/1
  HwModeRegister254/1 -> _adder_MultiplyAdd75/2
  HwModeRegister255/1 -> _adder_MultiplyAdd75/3
  _adder_MultiplyAdd76/1 -> PipelineRegister99/1
  HwModeRegister256/1 -> _adder_MultiplyAdd76/1
  HwModeRegister257/1 -> _adder_MultiplyAdd76/2
  HwModeRegister258/1 -> _adder_MultiplyAdd76/3
  _adder_MultiplyAdd77/1 -> PipelineRegister100/1
  HwModeRegister259/1 -> _adder_MultiplyAdd77/1
  HwModeRegister260/1 -> _adder_MultiplyAdd77/2
  HwModeRegister261/1 -> _adder_MultiplyAdd77/3
  _adder_MultiplyAdd78/1 -> PipelineRegister101/1
  HwModeRegister262/1 -> _adder_MultiplyAdd78/1
  HwModeRegister263/1 -> _adder_MultiplyAdd78/2
  HwModeRegister264/1 -> _adder_MultiplyAdd78/3
  _adder_MultiplyAdd79/1 -> PipelineRegister102/1
  HwModeRegister265/1 -> _adder_MultiplyAdd79/1
  HwModeRegister266/1 -> _adder_MultiplyAdd79/2
  HwModeRegister267/1 -> _adder_MultiplyAdd79/3
  _adder_MultiplyAdd80/1 -> PipelineRegister103/1
  HwModeRegister268/1 -> _adder_MultiplyAdd80/1
  HwModeRegister269/1 -> _adder_MultiplyAdd80/2
  HwModeRegister270/1 -> _adder_MultiplyAdd80/3
  Gain2/1 -> PipelineRegister104/1
  HwModeRegister271/1 -> Gain2/1
  HwModeRegister272/1 -> Gain2/2
  Gain21/1 -> PipelineRegister105/1
  HwModeRegister273/1 -> Gain21/1
  HwModeRegister274/1 -> Gain21/2
  Gain22/1 -> PipelineRegister106/1
  HwModeRegister275/1 -> Gain22/1
  HwModeRegister276/1 -> Gain22/2
  Gain/1 -> PipelineRegister107/1
  HwModeRegister277/1 -> Gain/1
  HwModeRegister278/1 -> Gain/2
  Product/1 -> PipelineRegister108/1
  HwModeRegister279/1 -> Product/1
  HwModeRegister280/1 -> Product/2
  Product1/1 -> PipelineRegister109/1
  HwModeRegister281/1 -> Product1/1
  HwModeRegister282/1 -> Product1/2
  Product2/1 -> PipelineRegister110/1
  HwModeRegister283/1 -> Product2/1
  HwModeRegister284/1 -> Product2/2
  Product3/1 -> PipelineRegister111/1
  HwModeRegister285/1 -> Product3/1
  HwModeRegister286/1 -> Product3/2
  Product4/1 -> PipelineRegister112/1
  HwModeRegister287/1 -> Product4/1
  HwModeRegister288/1 -> Product4/2
  Product5/1 -> PipelineRegister113/1
  HwModeRegister289/1 -> Product5/1
  HwModeRegister290/1 -> Product5/2
  Product6/1 -> PipelineRegister114/1
  HwModeRegister291/1 -> Product6/1
  HwModeRegister292/1 -> Product6/2
  Product7/1 -> PipelineRegister115/1
  HwModeRegister293/1 -> Product7/1
  HwModeRegister294/1 -> Product7/2
  Product8/1 -> PipelineRegister116/1
  HwModeRegister295/1 -> Product8/1
  HwModeRegister296/1 -> Product8/2
  Product9/1 -> PipelineRegister117/1
  HwModeRegister297/1 -> Product9/1
  HwModeRegister298/1 -> Product9/2
  Product10/1 -> PipelineRegister118/1
  HwModeRegister299/1 -> Product10/1
  HwModeRegister300/1 -> Product10/2
  Product11/1 -> PipelineRegister119/1
  HwModeRegister301/1 -> Product11/1
  HwModeRegister302/1 -> Product11/2
